simulink model "model"  (R2016a)
(part 10 of 11)

  548_CN_137197826_380000_CN_52983550_380000/LConn2 -- T_137197826_380000;220000;110000_Neuenhagen/LConn2 -- 517_CN_137197826_380000_CN_20562114_380000/LConn2 -- 495;_496_CN_137197826_380000_CN_22973070_380000/LConn2 -- 548_CN_137197826_380000_CN_23025610_380000/LConn2 -- 517_CN_137197826_380000_CN_29877599_380000/RConn2
  548_CN_137197826_380000_CN_52983550_380000/LConn3 -- T_137197826_380000;220000;110000_Neuenhagen/LConn3 -- 517_CN_137197826_380000_CN_20562114_380000/LConn3 -- 495;_496_CN_137197826_380000_CN_22973070_380000/LConn3 -- 548_CN_137197826_380000_CN_23025610_380000/LConn3 -- 517_CN_137197826_380000_CN_29877599_380000/RConn3
  T_52983550_380000;110000_Eisenhüttenstadt/LConn1 -- 548_CN_137197826_380000_CN_52983550_380000/RConn1
  T_52983550_380000;110000_Eisenhüttenstadt/LConn2 -- 548_CN_137197826_380000_CN_52983550_380000/RConn2
  T_52983550_380000;110000_Eisenhüttenstadt/LConn3 -- 548_CN_137197826_380000_CN_52983550_380000/RConn3
  548_CN_137197826_380000_CN_23025610_380000/RConn1 -- T_23025610_380000;110000_Umspannwerk_Preilack/LConn1 -- 561_CN_30164703_380000_CN_23025610_380000/LConn1 -- _CN_156683994_380000_CN_23025610_380000/LConn1 -- 559_CN_157328339_380000_CN_23025610_380000/LConn1 -- _CN_23025610_380000_CN11341038/LConn1
  548_CN_137197826_380000_CN_23025610_380000/RConn2 -- T_23025610_380000;110000_Umspannwerk_Preilack/LConn2 -- 561_CN_30164703_380000_CN_23025610_380000/LConn2 -- _CN_156683994_380000_CN_23025610_380000/LConn2 -- 559_CN_157328339_380000_CN_23025610_380000/LConn2 -- _CN_23025610_380000_CN11341038/LConn2
  548_CN_137197826_380000_CN_23025610_380000/RConn3 -- T_23025610_380000;110000_Umspannwerk_Preilack/LConn3 -- 561_CN_30164703_380000_CN_23025610_380000/LConn3 -- _CN_156683994_380000_CN_23025610_380000/LConn3 -- 559_CN_157328339_380000_CN_23025610_380000/LConn3 -- _CN_23025610_380000_CN11341038/LConn3
  T_20562114_380000;110000_Umspannwerk_Malchow/LConn1 -- 517_CN_137197826_380000_CN_20562114_380000/RConn1
  T_20562114_380000;110000_Umspannwerk_Malchow/LConn2 -- 517_CN_137197826_380000_CN_20562114_380000/RConn2
  T_20562114_380000;110000_Umspannwerk_Malchow/LConn3 -- 517_CN_137197826_380000_CN_20562114_380000/RConn3
  495;_496_CN_137197826_380000_CN_22973070_380000/RConn1 -- T_22973070_380000;220000;110000_Umspannwerk_Marzahn/LConn1 -- _CN_22973070_380000_CN_30954714_380000/LConn1
  495;_496_CN_137197826_380000_CN_22973070_380000/RConn2 -- T_22973070_380000;220000;110000_Umspannwerk_Marzahn/LConn2 -- _CN_22973070_380000_CN_30954714_380000/LConn2
  495;_496_CN_137197826_380000_CN_22973070_380000/RConn3 -- T_22973070_380000;220000;110000_Umspannwerk_Marzahn/LConn3 -- _CN_22973070_380000_CN_30954714_380000/LConn3
  526_CN_29331499_220000_CN_27149550_220000/LConn1 -- T_29331499_380000;220000;110000_Thyrow/RConn1 -- 302_CN_29331499_220000_CN_22973070_220000/LConn1 -- 302_CN_29331499_220000_CN_22973052_220000/LConn1
  526_CN_29331499_220000_CN_27149550_220000/LConn2 -- T_29331499_380000;220000;110000_Thyrow/RConn2 -- 302_CN_29331499_220000_CN_22973070_220000/LConn2 -- 302_CN_29331499_220000_CN_22973052_220000/LConn2
  526_CN_29331499_220000_CN_27149550_220000/LConn3 -- T_29331499_380000;220000;110000_Thyrow/RConn3 -- 302_CN_29331499_220000_CN_22973070_220000/LConn3 -- 302_CN_29331499_220000_CN_22973052_220000/LConn3
  526_CN_29331499_220000_CN_27149550_220000/RConn1 -- T_27149550_380000;220000;110000_Wustermark/RConn1 -- 294_CN_27149550_220000_CN215092049/RConn1 -- 294_CN_27149550_220000_CN_30309989_220000/LConn1 -- 324_CN_40621568_220000_CN_27149550_220000/LConn1
  526_CN_29331499_220000_CN_27149550_220000/RConn2 -- T_27149550_380000;220000;110000_Wustermark/RConn2 -- 294_CN_27149550_220000_CN215092049/RConn2 -- 294_CN_27149550_220000_CN_30309989_220000/LConn2 -- 324_CN_40621568_220000_CN_27149550_220000/LConn2
  526_CN_29331499_220000_CN_27149550_220000/RConn3 -- T_27149550_380000;220000;110000_Wustermark/RConn3 -- 294_CN_27149550_220000_CN215092049/RConn3 -- 294_CN_27149550_220000_CN_30309989_220000/LConn3 -- 324_CN_40621568_220000_CN_27149550_220000/LConn3
  302_CN_29331499_220000_CN_22973070_220000/RConn1 -- T_22973070_380000;220000;110000_Umspannwerk_Marzahn/RConn1 -- _CN_285823537_220000_CN_22973070_220000/LConn1
  302_CN_29331499_220000_CN_22973070_220000/RConn2 -- T_22973070_380000;220000;110000_Umspannwerk_Marzahn/RConn2 -- _CN_285823537_220000_CN_22973070_220000/LConn2
  302_CN_29331499_220000_CN_22973070_220000/RConn3 -- T_22973070_380000;220000;110000_Umspannwerk_Marzahn/RConn3 -- _CN_285823537_220000_CN_22973070_220000/LConn3
  T_22973052_220000;110000_Umspannwerk_Wuhlheide/LConn1 -- 302_CN_29331499_220000_CN_22973052_220000/RConn1
  T_22973052_220000;110000_Umspannwerk_Wuhlheide/LConn2 -- 302_CN_29331499_220000_CN_22973052_220000/RConn2
  T_22973052_220000;110000_Umspannwerk_Wuhlheide/LConn3 -- 302_CN_29331499_220000_CN_22973052_220000/RConn3
  T_29331499_380000;220000;110000_Thyrow/LConn1 -- 522_CN_29331499_380000_CN_27149550_380000/LConn1
  T_29331499_380000;220000;110000_Thyrow/LConn2 -- 522_CN_29331499_380000_CN_27149550_380000/LConn2
  T_29331499_380000;220000;110000_Thyrow/LConn3 -- 522_CN_29331499_380000_CN_27149550_380000/LConn3
  522_CN_29331499_380000_CN_27149550_380000/RConn1 -- T_27149550_380000;220000;110000_Wustermark/LConn1 -- 493_CN_26472665_380000_CN_27149550_380000/LConn1
  522_CN_29331499_380000_CN_27149550_380000/RConn2 -- T_27149550_380000;220000;110000_Wustermark/LConn2 -- 493_CN_26472665_380000_CN_27149550_380000/LConn2
  522_CN_29331499_380000_CN_27149550_380000/RConn3 -- T_27149550_380000;220000;110000_Wustermark/LConn3 -- 493_CN_26472665_380000_CN_27149550_380000/LConn3
  Helmstedt_380_kV_CN_26474759_380000_CN_24258096_380000/RConn1 -- T_26474759_380000;110000_Umspannwerk_Helmstedt/LConn1 -- Helmstedt_380_kV_CN_26474759_380000_CN_26472665_380000/LConn1 -- Leitung_3845_(System_301)_CN_26474759_380000_CN_199382606_380000/LConn1
  Helmstedt_380_kV_CN_26474759_380000_CN_24258096_380000/RConn2 -- T_26474759_380000;110000_Umspannwerk_Helmstedt/LConn2 -- Helmstedt_380_kV_CN_26474759_380000_CN_26472665_380000/LConn2 -- Leitung_3845_(System_301)_CN_26474759_380000_CN_199382606_380000/LConn2
  Helmstedt_380_kV_CN_26474759_380000_CN_24258096_380000/RConn3 -- T_26474759_380000;110000_Umspannwerk_Helmstedt/LConn3 -- Helmstedt_380_kV_CN_26474759_380000_CN_26472665_380000/LConn3 -- Leitung_3845_(System_301)_CN_26474759_380000_CN_199382606_380000/LConn3
  T_199382606__/LConn1 -- Leitung_3845_(System_301)_CN_26474759_380000_CN_199382606_380000/RConn1
  T_199382606__/LConn2 -- Leitung_3845_(System_301)_CN_26474759_380000_CN_199382606_380000/RConn2
  T_199382606__/LConn3 -- Leitung_3845_(System_301)_CN_26474759_380000_CN_199382606_380000/RConn3
  Helmstedt_380_kV_CN_26474759_380000_CN_26472665_380000/RConn1 -- T_26472665_380000;220000_Umspannwerk_Wolmirstedt/LConn1 -- 493_CN_26472665_380000_CN_30132758_380000/LConn1 -- 493_CN_26472665_380000_CN_27149550_380000/RConn1 -- 438_CN_26472665_380000_CN_156683994_380000/LConn1 -- 536_CN_26472665_380000_CN_32690742_380000/LConn1 -- 536_CN_26472665_380000_CN_29713902_380000/LConn1 -- 490_CN_26472665_380000_CN_33169401_380000/RConn1
  Helmstedt_380_kV_CN_26474759_380000_CN_26472665_380000/RConn2 -- T_26472665_380000;220000_Umspannwerk_Wolmirstedt/LConn2 -- 493_CN_26472665_380000_CN_30132758_380000/LConn2 -- 493_CN_26472665_380000_CN_27149550_380000/RConn2 -- 438_CN_26472665_380000_CN_156683994_380000/LConn2 -- 536_CN_26472665_380000_CN_32690742_380000/LConn2 -- 536_CN_26472665_380000_CN_29713902_380000/LConn2 -- 490_CN_26472665_380000_CN_33169401_380000/RConn2
  Helmstedt_380_kV_CN_26474759_380000_CN_26472665_380000/RConn3 -- T_26472665_380000;220000_Umspannwerk_Wolmirstedt/LConn3 -- 493_CN_26472665_380000_CN_30132758_380000/LConn3 -- 493_CN_26472665_380000_CN_27149550_380000/RConn3 -- 438_CN_26472665_380000_CN_156683994_380000/LConn3 -- 536_CN_26472665_380000_CN_32690742_380000/LConn3 -- 536_CN_26472665_380000_CN_29713902_380000/LConn3 -- 490_CN_26472665_380000_CN_33169401_380000/RConn3
  _CN_29344008_220000_CN_151765495_220000/RConn1 -- T_151765495_220000_Götzdorf/LConn1 -- _CN_151765495_220000_CN_229500139_220000/LConn1
  _CN_29344008_220000_CN_151765495_220000/RConn2 -- T_151765495_220000_Götzdorf/LConn2 -- _CN_151765495_220000_CN_229500139_220000/LConn2
  _CN_29344008_220000_CN_151765495_220000/RConn3 -- T_151765495_220000_Götzdorf/LConn3 -- _CN_151765495_220000_CN_229500139_220000/LConn3
  T_25306938_220000;110000_Kummerfeld/LConn1 -- _CN_29344008_220000_CN_25306938_220000/RConn1
  T_25306938_220000;110000_Kummerfeld/LConn2 -- _CN_29344008_220000_CN_25306938_220000/RConn2
  T_25306938_220000;110000_Kummerfeld/LConn3 -- _CN_29344008_220000_CN_25306938_220000/RConn3
  _CN_25557259_380000_CN_43688805_380000/LConn1 -- T_25557259__/LConn1 -- _CN_25557259_380000_CN_143854536_380000/LConn1 -- _CN_25557259_380000_CN_25557397_380000/LConn1 -- _CN_25557259_380000_CN_145002769_380000/LConn1 -- _CN_25557259_380000_CN_143903369_380000/LConn1 -- _CN_25557259_380000_CN_153328698_380000/LConn1 -- _CN_25557259_380000_CN89183108/LConn1
  _CN_25557259_380000_CN_43688805_380000/LConn2 -- T_25557259__/LConn2 -- _CN_25557259_380000_CN_143854536_380000/LConn2 -- _CN_25557259_380000_CN_25557397_380000/LConn2 -- _CN_25557259_380000_CN_145002769_380000/LConn2 -- _CN_25557259_380000_CN_143903369_380000/LConn2 -- _CN_25557259_380000_CN_153328698_380000/LConn2 -- _CN_25557259_380000_CN89183108/LConn2
  _CN_25557259_380000_CN_43688805_380000/LConn3 -- T_25557259__/LConn3 -- _CN_25557259_380000_CN_143854536_380000/LConn3 -- _CN_25557259_380000_CN_25557397_380000/LConn3 -- _CN_25557259_380000_CN_145002769_380000/LConn3 -- _CN_25557259_380000_CN_143903369_380000/LConn3 -- _CN_25557259_380000_CN_153328698_380000/LConn3 -- _CN_25557259_380000_CN89183108/LConn3
  _CN_25557259_380000_CN_43688805_380000/RConn1 -- T_43688805_380000;220000;110000_380kV_Umspannwerk_Pulverdingen/LConn1 -- Philippsburg___Pulverdingen_CN_43688805_380000_CN_254326606_380000/LConn1 -- Philippsburg___Pulverdingen_CN_43688805_380000_CN_154110135_380000/RConn1 -- 380_kV_CN_26260052_380000_CN_43688805_380000/LConn1 -- 2x_380_kV_CN_43688805_380000_CN_26814283_380000/LConn1
  _CN_25557259_380000_CN_43688805_380000/RConn2 -- T_43688805_380000;220000;110000_380kV_Umspannwerk_Pulverdingen/LConn2 -- Philippsburg___Pulverdingen_CN_43688805_380000_CN_254326606_380000/LConn2 -- Philippsburg___Pulverdingen_CN_43688805_380000_CN_154110135_380000/RConn2 -- 380_kV_CN_26260052_380000_CN_43688805_380000/LConn2 -- 2x_380_kV_CN_43688805_380000_CN_26814283_380000/LConn2
  _CN_25557259_380000_CN_43688805_380000/RConn3 -- T_43688805_380000;220000;110000_380kV_Umspannwerk_Pulverdingen/LConn3 -- Philippsburg___Pulverdingen_CN_43688805_380000_CN_254326606_380000/LConn3 -- Philippsburg___Pulverdingen_CN_43688805_380000_CN_154110135_380000/RConn3 -- 380_kV_CN_26260052_380000_CN_43688805_380000/LConn3 -- 2x_380_kV_CN_43688805_380000_CN_26814283_380000/LConn3
  _CN_25557259_380000_CN89183108/RConn1 -- G_89183108_Heizkraftwerk_Heilbronn/RConn1 -- _CN_25557397_220000_CN89183108/RConn1
  _CN_25557259_380000_CN89183108/RConn2 -- G_89183108_Heizkraftwerk_Heilbronn/RConn2 -- _CN_25557397_220000_CN89183108/RConn2
  _CN_25557259_380000_CN89183108/RConn3 -- G_89183108_Heizkraftwerk_Heilbronn/RConn3 -- _CN_25557397_220000_CN89183108/RConn3
  _CN_25557259_380000_CN_143854536_380000/RConn1 -- T_143854536_380000;110000_Umspannwerk_Kupferzell/LConn1 -- _CN_145002769_380000_CN_143854536_380000/LConn1 -- Goldshöfe___Kupferzell_CN_42050342_380000_CN_143854536_380000/RConn1
  _CN_25557259_380000_CN_143854536_380000/RConn2 -- T_143854536_380000;110000_Umspannwerk_Kupferzell/LConn2 -- _CN_145002769_380000_CN_143854536_380000/LConn2 -- Goldshöfe___Kupferzell_CN_42050342_380000_CN_143854536_380000/RConn2
  _CN_25557259_380000_CN_143854536_380000/RConn3 -- T_143854536_380000;110000_Umspannwerk_Kupferzell/LConn3 -- _CN_145002769_380000_CN_143854536_380000/LConn3 -- Goldshöfe___Kupferzell_CN_42050342_380000_CN_143854536_380000/RConn3
  T_25557397_380000;220000;110000_380_kV_Umspannwerk_Großgartach/LConn1 -- _CN_25557259_380000_CN_25557397_380000/RConn1
  T_25557397_380000;220000;110000_380_kV_Umspannwerk_Großgartach/LConn2 -- _CN_25557259_380000_CN_25557397_380000/RConn2
  T_25557397_380000;220000;110000_380_kV_Umspannwerk_Großgartach/LConn3 -- _CN_25557259_380000_CN_25557397_380000/RConn3
  _CN_25557259_380000_CN_145002769_380000/RConn1 -- T_145002769_380000;110000_Umspannwerk_Höpfingen/LConn1 -- _CN_145002769_380000_CN_108797675_380000/RConn1 -- _CN_145002769_380000_CN_143854536_380000/RConn1
  _CN_25557259_380000_CN_145002769_380000/RConn2 -- T_145002769_380000;110000_Umspannwerk_Höpfingen/LConn2 -- _CN_145002769_380000_CN_108797675_380000/RConn2 -- _CN_145002769_380000_CN_143854536_380000/RConn2
  _CN_25557259_380000_CN_145002769_380000/RConn3 -- T_145002769_380000;110000_Umspannwerk_Höpfingen/LConn3 -- _CN_145002769_380000_CN_108797675_380000/RConn3 -- _CN_145002769_380000_CN_143854536_380000/RConn3
  _CN_25557259_380000_CN_143903369_380000/RConn1 -- T_143903369_380000;220000;110000_Umspannwerk_Hüffenhardt/LConn1 -- Elsenz_CN_143903369_380000_CN_46584363_380000/LConn1 -- Elsenz_CN_143903369_380000_CN_154110135_380000/RConn1 -- Elsenz_CN_143903369_380000_CN_207248812_380000/LConn1
  _CN_25557259_380000_CN_143903369_380000/RConn2 -- T_143903369_380000;220000;110000_Umspannwerk_Hüffenhardt/LConn2 -- Elsenz_CN_143903369_380000_CN_46584363_380000/LConn2 -- Elsenz_CN_143903369_380000_CN_154110135_380000/RConn2 -- Elsenz_CN_143903369_380000_CN_207248812_380000/LConn2
  _CN_25557259_380000_CN_143903369_380000/RConn3 -- T_143903369_380000;220000;110000_Umspannwerk_Hüffenhardt/LConn3 -- Elsenz_CN_143903369_380000_CN_46584363_380000/LConn3 -- Elsenz_CN_143903369_380000_CN_154110135_380000/RConn3 -- Elsenz_CN_143903369_380000_CN_207248812_380000/LConn3
  _CN_25557259_380000_CN_153328698_380000/RConn1 -- T_153328698_380000_Gemeinschaftskraftwerk_Neckarwestheim_2/LConn1 -- _CN_147878692_380000_CN_153328698_380000/LConn1 -- _CN_153328698_380000_CN23547196/RConn1
  _CN_25557259_380000_CN_153328698_380000/RConn2 -- T_153328698_380000_Gemeinschaftskraftwerk_Neckarwestheim_2/LConn2 -- _CN_147878692_380000_CN_153328698_380000/LConn2 -- _CN_153328698_380000_CN23547196/RConn2
  _CN_25557259_380000_CN_153328698_380000/RConn3 -- T_153328698_380000_Gemeinschaftskraftwerk_Neckarwestheim_2/LConn3 -- _CN_147878692_380000_CN_153328698_380000/LConn3 -- _CN_153328698_380000_CN23547196/RConn3
  T_169244940_380000_Station_Kelsterbach/LConn1 -- _CN_169244940_380000_CN_55730023_380000/LConn1
  T_169244940_380000_Station_Kelsterbach/LConn2 -- _CN_169244940_380000_CN_55730023_380000/LConn2
  T_169244940_380000_Station_Kelsterbach/LConn3 -- _CN_169244940_380000_CN_55730023_380000/LConn3
  _CN_169244940_380000_CN_55730023_380000/RConn1 -- T_55730023_380000_Kabeleinführung_380_kV/LConn1 -- 2_x_380_kV;_3_x_220_kV_CN_23284340_380000_CN_55730023_380000/LConn1
  _CN_169244940_380000_CN_55730023_380000/RConn2 -- T_55730023_380000_Kabeleinführung_380_kV/LConn2 -- 2_x_380_kV;_3_x_220_kV_CN_23284340_380000_CN_55730023_380000/LConn2
  _CN_169244940_380000_CN_55730023_380000/RConn3 -- T_55730023_380000_Kabeleinführung_380_kV/LConn3 -- 2_x_380_kV;_3_x_220_kV_CN_23284340_380000_CN_55730023_380000/LConn3
  T_29417741_220000_Umspannwerk_Regensburg/LConn1 -- Regensburg___Schwandorf_CN_29417741_220000_CN_28956649_220000/RConn1
  T_29417741_220000_Umspannwerk_Regensburg/LConn2 -- Regensburg___Schwandorf_CN_29417741_220000_CN_28956649_220000/RConn2
  T_29417741_220000_Umspannwerk_Regensburg/LConn3 -- Regensburg___Schwandorf_CN_29417741_220000_CN_28956649_220000/RConn3
  501_CN_28729619_380000_CN_25526912_380000/LConn1 -- T_28729619_380000_Umspannwerk_Schönewalde/LConn1 -- 501_CN_28729619_380000_CN_156683994_380000/LConn1 -- 501_CN_28729619_380000_CN_29713902_380000/LConn1
  501_CN_28729619_380000_CN_25526912_380000/LConn2 -- T_28729619_380000_Umspannwerk_Schönewalde/LConn2 -- 501_CN_28729619_380000_CN_156683994_380000/LConn2 -- 501_CN_28729619_380000_CN_29713902_380000/LConn2
  501_CN_28729619_380000_CN_25526912_380000/LConn3 -- T_28729619_380000_Umspannwerk_Schönewalde/LConn3 -- 501_CN_28729619_380000_CN_156683994_380000/LConn3 -- 501_CN_28729619_380000_CN_29713902_380000/LConn3
  T_25526912_380000;110000_Umspannwerk_Marke/LConn1 -- 501_CN_28729619_380000_CN_25526912_380000/RConn1
  T_25526912_380000;110000_Umspannwerk_Marke/LConn2 -- 501_CN_28729619_380000_CN_25526912_380000/RConn2
  T_25526912_380000;110000_Umspannwerk_Marke/LConn3 -- 501_CN_28729619_380000_CN_25526912_380000/RConn3
  501_CN_28729619_380000_CN_29713902_380000/RConn1 -- T_29713902_380000;110000_Umspannwerk_Lauchstädt/LConn1 -- _CN_29713902_380000_CN218161891/LConn1 -- _CN_143882655_380000_CN_29713902_380000/RConn1 -- 536_CN_26472665_380000_CN_29713902_380000/RConn1
  501_CN_28729619_380000_CN_29713902_380000/RConn2 -- T_29713902_380000;110000_Umspannwerk_Lauchstädt/LConn2 -- _CN_29713902_380000_CN218161891/LConn2 -- _CN_143882655_380000_CN_29713902_380000/RConn2 -- 536_CN_26472665_380000_CN_29713902_380000/RConn2
  501_CN_28729619_380000_CN_29713902_380000/RConn3 -- T_29713902_380000;110000_Umspannwerk_Lauchstädt/LConn3 -- _CN_29713902_380000_CN218161891/LConn3 -- _CN_143882655_380000_CN_29713902_380000/RConn3 -- 536_CN_26472665_380000_CN_29713902_380000/RConn3
  501_CN_28729619_380000_CN_156683994_380000/RConn1 -- T_156683994_380000;110000_Umspannwerk_Ragow/LConn1 -- _CN_156683994_380000_CN_23025610_380000/RConn1 -- 438_CN_26472665_380000_CN_156683994_380000/RConn1 -- 561_Streumen_CN_156683994_380000_CN_157328339_380000/LConn1
  501_CN_28729619_380000_CN_156683994_380000/RConn2 -- T_156683994_380000;110000_Umspannwerk_Ragow/LConn2 -- _CN_156683994_380000_CN_23025610_380000/RConn2 -- 438_CN_26472665_380000_CN_156683994_380000/RConn2 -- 561_Streumen_CN_156683994_380000_CN_157328339_380000/LConn2
  501_CN_28729619_380000_CN_156683994_380000/RConn3 -- T_156683994_380000;110000_Umspannwerk_Ragow/LConn3 -- _CN_156683994_380000_CN_23025610_380000/RConn3 -- 438_CN_26472665_380000_CN_156683994_380000/RConn3 -- 561_Streumen_CN_156683994_380000_CN_157328339_380000/LConn3
  T_53378027_380000;110000_Umspannwerk_Lechhausen;_Übernahmestation_Lechhausen/LConn1 -- _CN_30613895_380000_CN_53378027_380000/RConn1
  T_53378027_380000;110000_Umspannwerk_Lechhausen;_Übernahmestation_Lechhausen/LConn2 -- _CN_30613895_380000_CN_53378027_380000/RConn2
  T_53378027_380000;110000_Umspannwerk_Lechhausen;_Übernahmestation_Lechhausen/LConn3 -- _CN_30613895_380000_CN_53378027_380000/RConn3
  _CN_30613895_380000_CN_24652261_380000/RConn1 -- T_24652261_380000_Station_Meitingen/LConn1 -- Meitingen_Nord;_Süd_CN_24652261_380000_CN_85523877_380000/RConn1 -- Meitingen_Nord;_Süd_CN_24652261_380000_CN_88945213_380000/LConn1 -- _CN_24652261_380000_CN_76246159_380000/LConn1 -- MEI_OBA_CN_24652261_380000_CN_18629425_380000/RConn1
  _CN_30613895_380000_CN_24652261_380000/RConn2 -- T_24652261_380000_Station_Meitingen/LConn2 -- Meitingen_Nord;_Süd_CN_24652261_380000_CN_85523877_380000/RConn2 -- Meitingen_Nord;_Süd_CN_24652261_380000_CN_88945213_380000/LConn2 -- _CN_24652261_380000_CN_76246159_380000/LConn2 -- MEI_OBA_CN_24652261_380000_CN_18629425_380000/RConn2
  _CN_30613895_380000_CN_24652261_380000/RConn3 -- T_24652261_380000_Station_Meitingen/LConn3 -- Meitingen_Nord;_Süd_CN_24652261_380000_CN_85523877_380000/RConn3 -- Meitingen_Nord;_Süd_CN_24652261_380000_CN_88945213_380000/LConn3 -- _CN_24652261_380000_CN_76246159_380000/LConn3 -- MEI_OBA_CN_24652261_380000_CN_18629425_380000/RConn3
  380_kV_Gilzem_Ost;_Uchtelfangen_Ost_CN_42097854_380000_CN_54359256_380000/LConn1 -- T_42097854_380000;110000_Station_Osburg/LConn1 -- 380_kV_Gilzem_Ost;_Uchtelfangen_Ost_CN_42097854_380000_CN_151967290_380000/LConn1
  380_kV_Gilzem_Ost;_Uchtelfangen_Ost_CN_42097854_380000_CN_54359256_380000/LConn2 -- T_42097854_380000;110000_Station_Osburg/LConn2 -- 380_kV_Gilzem_Ost;_Uchtelfangen_Ost_CN_42097854_380000_CN_151967290_380000/LConn2
  380_kV_Gilzem_Ost;_Uchtelfangen_Ost_CN_42097854_380000_CN_54359256_380000/LConn3 -- T_42097854_380000;110000_Station_Osburg/LConn3 -- 380_kV_Gilzem_Ost;_Uchtelfangen_Ost_CN_42097854_380000_CN_151967290_380000/LConn3
  380_kV_Gilzem_Ost;_Uchtelfangen_Ost_CN_42097854_380000_CN_54359256_380000/RConn1 -- T_54359256_380000;220000;110000_Umspannwerk_Uchtelfangen/LConn1 -- _CN_54359256_380000_CN115145869/LConn1 -- _CN_152261133_380000_CN_54359256_380000/RConn1
  380_kV_Gilzem_Ost;_Uchtelfangen_Ost_CN_42097854_380000_CN_54359256_380000/RConn2 -- T_54359256_380000;220000;110000_Umspannwerk_Uchtelfangen/LConn2 -- _CN_54359256_380000_CN115145869/LConn2 -- _CN_152261133_380000_CN_54359256_380000/RConn2
  380_kV_Gilzem_Ost;_Uchtelfangen_Ost_CN_42097854_380000_CN_54359256_380000/RConn3 -- T_54359256_380000;220000;110000_Umspannwerk_Uchtelfangen/LConn3 -- _CN_54359256_380000_CN115145869/LConn3 -- _CN_152261133_380000_CN_54359256_380000/RConn3
  380_kV_Gilzem_Ost;_Uchtelfangen_Ost_CN_42097854_380000_CN_151967290_380000/RConn1 -- T_151967290_380000;220000;110000_Station_Niederstedem/LConn1 -- _CN_151967290_380000_CN_32675761_380000/LConn1 -- _CN_151967290_380000_CN_26593929_380000/RConn1
  380_kV_Gilzem_Ost;_Uchtelfangen_Ost_CN_42097854_380000_CN_151967290_380000/RConn2 -- T_151967290_380000;220000;110000_Station_Niederstedem/LConn2 -- _CN_151967290_380000_CN_32675761_380000/LConn2 -- _CN_151967290_380000_CN_26593929_380000/RConn2
  380_kV_Gilzem_Ost;_Uchtelfangen_Ost_CN_42097854_380000_CN_151967290_380000/RConn3 -- T_151967290_380000;220000;110000_Station_Niederstedem/LConn3 -- _CN_151967290_380000_CN_32675761_380000/LConn3 -- _CN_151967290_380000_CN_26593929_380000/RConn3
  220kV_Welper_Ost+ANK_CN_156973363_220000_CN_63114179_220000/LConn1 -- T_156973363_220000_Station_Welper/LConn1 -- 220kV_Welper_Ost+ANK_CN_156973363_220000_CN_86163350_220000/LConn1 -- 220kV_Welper_Ost+ANK_CN_156973363_220000_CN_68549340_220000/RConn1
  220kV_Welper_Ost+ANK_CN_156973363_220000_CN_63114179_220000/LConn2 -- T_156973363_220000_Station_Welper/LConn2 -- 220kV_Welper_Ost+ANK_CN_156973363_220000_CN_86163350_220000/LConn2 -- 220kV_Welper_Ost+ANK_CN_156973363_220000_CN_68549340_220000/RConn2
  220kV_Welper_Ost+ANK_CN_156973363_220000_CN_63114179_220000/LConn3 -- T_156973363_220000_Station_Welper/LConn3 -- 220kV_Welper_Ost+ANK_CN_156973363_220000_CN_86163350_220000/LConn3 -- 220kV_Welper_Ost+ANK_CN_156973363_220000_CN_68549340_220000/RConn3
  T_63114179_380000;220000;110000_Station_Hattingen/RConn1 -- 220kV_Welper_Ost+ANK_CN_156973363_220000_CN_63114179_220000/RConn1
  T_63114179_380000;220000;110000_Station_Hattingen/RConn2 -- 220kV_Welper_Ost+ANK_CN_156973363_220000_CN_63114179_220000/RConn2
  T_63114179_380000;220000;110000_Station_Hattingen/RConn3 -- 220kV_Welper_Ost+ANK_CN_156973363_220000_CN_63114179_220000/RConn3
  T_86163350_220000_UW_Stahlwerk_ThyssenKrupp_Nirosta/LConn1 -- 220kV_Welper_Ost+ANK_CN_156973363_220000_CN_86163350_220000/RConn1
  T_86163350_220000_UW_Stahlwerk_ThyssenKrupp_Nirosta/LConn2 -- 220kV_Welper_Ost+ANK_CN_156973363_220000_CN_86163350_220000/RConn2
  T_86163350_220000_UW_Stahlwerk_ThyssenKrupp_Nirosta/LConn3 -- 220kV_Welper_Ost+ANK_CN_156973363_220000_CN_86163350_220000/RConn3
  T_153334076__/LConn1 -- _CN_153334076_220000_CN23547196/RConn1
  T_153334076__/LConn2 -- _CN_153334076_220000_CN23547196/RConn2
  T_153334076__/LConn3 -- _CN_153334076_220000_CN23547196/RConn3
  329_CN_35102433_220000_CN_26472665_220000/LConn1 -- T_35102433_220000;110000_Magdeburg_(50Hertz)/LConn1 -- 335_CN_35102433_220000_CN_35137205_220000/LConn1
  329_CN_35102433_220000_CN_26472665_220000/LConn2 -- T_35102433_220000;110000_Magdeburg_(50Hertz)/LConn2 -- 335_CN_35102433_220000_CN_35137205_220000/LConn2
  329_CN_35102433_220000_CN_26472665_220000/LConn3 -- T_35102433_220000;110000_Magdeburg_(50Hertz)/LConn3 -- 335_CN_35102433_220000_CN_35137205_220000/LConn3
  329_CN_35102433_220000_CN_26472665_220000/RConn1 -- T_26472665_380000;220000_Umspannwerk_Wolmirstedt/RConn1 -- 344_CN_26472665_220000_CN_35137205_220000/LConn1 -- L_26472665/LConn1
  329_CN_35102433_220000_CN_26472665_220000/RConn2 -- T_26472665_380000;220000_Umspannwerk_Wolmirstedt/RConn2 -- 344_CN_26472665_220000_CN_35137205_220000/LConn2 -- L_26472665/LConn2
  329_CN_35102433_220000_CN_26472665_220000/RConn3 -- T_26472665_380000;220000_Umspannwerk_Wolmirstedt/RConn3 -- 344_CN_26472665_220000_CN_35137205_220000/LConn3 -- L_26472665/LConn3
  335_CN_35102433_220000_CN_35137205_220000/RConn1 -- T_35137205_220000;110000_Umspannwerk_Förderstedt/LConn1 -- 344_CN_26472665_220000_CN_35137205_220000/RConn1
  335_CN_35102433_220000_CN_35137205_220000/RConn2 -- T_35137205_220000;110000_Umspannwerk_Förderstedt/LConn2 -- 344_CN_26472665_220000_CN_35137205_220000/RConn2
  335_CN_35102433_220000_CN_35137205_220000/RConn3 -- T_35137205_220000;110000_Umspannwerk_Förderstedt/LConn3 -- 344_CN_26472665_220000_CN_35137205_220000/RConn3
  _CN_91086220_220000_CN_24976300_220000/LConn1 -- T_91086220_220000_Umspannwerk_Simbach/LConn1 -- _CN_91086220_220000_CN_77694901_220000/LConn1 -- _CN_91086220_220000_CN167578660/RConn1
  _CN_91086220_220000_CN_24976300_220000/LConn2 -- T_91086220_220000_Umspannwerk_Simbach/LConn2 -- _CN_91086220_220000_CN_77694901_220000/LConn2 -- _CN_91086220_220000_CN167578660/RConn2
  _CN_91086220_220000_CN_24976300_220000/LConn3 -- T_91086220_220000_Umspannwerk_Simbach/LConn3 -- _CN_91086220_220000_CN_77694901_220000/LConn3 -- _CN_91086220_220000_CN167578660/RConn3
  _CN_91086220_220000_CN_24976300_220000/RConn1 -- T_24976300_380000;220000;110000_Umspannwerk_Pleinting/RConn1 -- Pleinting___Schwandorf_CN_24976300_220000_CN_28956649_220000/RConn1
  _CN_91086220_220000_CN_24976300_220000/RConn2 -- T_24976300_380000;220000;110000_Umspannwerk_Pleinting/RConn2 -- Pleinting___Schwandorf_CN_24976300_220000_CN_28956649_220000/RConn2
  _CN_91086220_220000_CN_24976300_220000/RConn3 -- T_24976300_380000;220000;110000_Umspannwerk_Pleinting/RConn3 -- Pleinting___Schwandorf_CN_24976300_220000_CN_28956649_220000/RConn3
  _CN_91086220_220000_CN_77694901_220000/RConn1 -- T_77694901_220000;110000_Umspannwerk_Altheim/LConn1 -- Altheim___Sittling_CN_24759324_220000_CN_77694901_220000/LConn1
  _CN_91086220_220000_CN_77694901_220000/RConn2 -- T_77694901_220000;110000_Umspannwerk_Altheim/LConn2 -- Altheim___Sittling_CN_24759324_220000_CN_77694901_220000/LConn2
  _CN_91086220_220000_CN_77694901_220000/RConn3 -- T_77694901_220000;110000_Umspannwerk_Altheim/LConn3 -- Altheim___Sittling_CN_24759324_220000_CN_77694901_220000/LConn3
  _CN_152924498_220000_CN152506744/RConn1 -- G_152506744_Großkraftwerk_Mannheim/RConn1 -- _CN_163093653_220000_CN152506744/LConn1
  _CN_152924498_220000_CN152506744/RConn2 -- G_152506744_Großkraftwerk_Mannheim/RConn2 -- _CN_163093653_220000_CN152506744/LConn2
  _CN_152924498_220000_CN152506744/RConn3 -- G_152506744_Großkraftwerk_Mannheim/RConn3 -- _CN_163093653_220000_CN152506744/LConn3
  220kV_Fichtenhain_West+Utfort_West_CN_93278553_220000_CN_24815262_220000/LConn1 -- T_93278553_220000;110000_Station_Edelstahl_Krefeld/LConn1 -- 220kV_Fichtenhain_West+Utfort_West_CN_93278553_220000_CN_24799890_220000/RConn1 -- 220kV_Fichtenhain_West+Utfort_West_CN_93278553_220000_CN_23380800_220000/LConn1 -- 220kV_Fichtenhain_West+Utfort_West_CN_93278553_220000_CN92877616/LConn1 -- 220kV_Fichtenhain_West+Utfort_West_CN_93278553_220000_CN_91854336_220000/RConn1 -- 220kV_Fichtenhain_West+Utfort_West_CN_93278553_220000_CN_24479984_220000/LConn1
  220kV_Fichtenhain_West+Utfort_West_CN_93278553_220000_CN_24815262_220000/LConn2 -- T_93278553_220000;110000_Station_Edelstahl_Krefeld/LConn2 -- 220kV_Fichtenhain_West+Utfort_West_CN_93278553_220000_CN_24799890_220000/RConn2 -- 220kV_Fichtenhain_West+Utfort_West_CN_93278553_220000_CN_23380800_220000/LConn2 -- 220kV_Fichtenhain_West+Utfort_West_CN_93278553_220000_CN92877616/LConn2 -- 220kV_Fichtenhain_West+Utfort_West_CN_93278553_220000_CN_91854336_220000/RConn2 -- 220kV_Fichtenhain_West+Utfort_West_CN_93278553_220000_CN_24479984_220000/LConn2
  220kV_Fichtenhain_West+Utfort_West_CN_93278553_220000_CN_24815262_220000/LConn3 -- T_93278553_220000;110000_Station_Edelstahl_Krefeld/LConn3 -- 220kV_Fichtenhain_West+Utfort_West_CN_93278553_220000_CN_24799890_220000/RConn3 -- 220kV_Fichtenhain_West+Utfort_West_CN_93278553_220000_CN_23380800_220000/LConn3 -- 220kV_Fichtenhain_West+Utfort_West_CN_93278553_220000_CN92877616/LConn3 -- 220kV_Fichtenhain_West+Utfort_West_CN_93278553_220000_CN_91854336_220000/RConn3 -- 220kV_Fichtenhain_West+Utfort_West_CN_93278553_220000_CN_24479984_220000/LConn3
  T_24815262_380000;220000;110000_Station_Dülken/LConn1 -- 220kV_Fichtenhain_West+Utfort_West_CN_93278553_220000_CN_24815262_220000/RConn1
  T_24815262_380000;220000;110000_Station_Dülken/LConn2 -- 220kV_Fichtenhain_West+Utfort_West_CN_93278553_220000_CN_24815262_220000/RConn2
  T_24815262_380000;220000;110000_Station_Dülken/LConn3 -- 220kV_Fichtenhain_West+Utfort_West_CN_93278553_220000_CN_24815262_220000/RConn3
  220kV_Fichtenhain_West+Utfort_West_CN_93278553_220000_CN_23380800_220000/RConn1 -- T_23380800_380000;220000;110000_Station_Utfort/RConn1 -- 220kV_Wesel_Ost_CN_24462426_220000_CN_23380800_220000/RConn1
  220kV_Fichtenhain_West+Utfort_West_CN_93278553_220000_CN_23380800_220000/RConn2 -- T_23380800_380000;220000;110000_Station_Utfort/RConn2 -- 220kV_Wesel_Ost_CN_24462426_220000_CN_23380800_220000/RConn2
  220kV_Fichtenhain_West+Utfort_West_CN_93278553_220000_CN_23380800_220000/RConn3 -- T_23380800_380000;220000;110000_Station_Utfort/RConn3 -- 220kV_Wesel_Ost_CN_24462426_220000_CN_23380800_220000/RConn3
  220kV_Fichtenhain_West+Utfort_West_CN_93278553_220000_CN92877616/RConn1 -- G_92877616_Kraftwerk_Huckingen/RConn1 -- _CN_92877610_220000_CN92877616/LConn1 -- _CN_92877635_220000_CN92877616/LConn1
  220kV_Fichtenhain_West+Utfort_West_CN_93278553_220000_CN92877616/RConn2 -- G_92877616_Kraftwerk_Huckingen/RConn2 -- _CN_92877610_220000_CN92877616/LConn2 -- _CN_92877635_220000_CN92877616/LConn2
  220kV_Fichtenhain_West+Utfort_West_CN_93278553_220000_CN92877616/RConn3 -- G_92877616_Kraftwerk_Huckingen/RConn3 -- _CN_92877610_220000_CN92877616/LConn3 -- _CN_92877635_220000_CN92877616/LConn3
  T_24479984_220000;110000_Uerdingen/LConn1 -- 220kV_Fichtenhain_West+Utfort_West_CN_93278553_220000_CN_24479984_220000/RConn1
  T_24479984_220000;110000_Uerdingen/LConn2 -- 220kV_Fichtenhain_West+Utfort_West_CN_93278553_220000_CN_24479984_220000/RConn2
  T_24479984_220000;110000_Uerdingen/LConn3 -- 220kV_Fichtenhain_West+Utfort_West_CN_93278553_220000_CN_24479984_220000/RConn3
  T_74893659_380000;110000_HGÜ_Baltic_Cable___Stromrichterstation_Herrenwyk/LConn1 -- _CN_74893659_380000_CN_74893662_380000/LConn1
  T_74893659_380000;110000_HGÜ_Baltic_Cable___Stromrichterstation_Herrenwyk/LConn2 -- _CN_74893659_380000_CN_74893662_380000/LConn2
  T_74893659_380000;110000_HGÜ_Baltic_Cable___Stromrichterstation_Herrenwyk/LConn3 -- _CN_74893659_380000_CN_74893662_380000/LConn3
  T_74893662_380000;220000;110000_Umspannwerk_Siems/LConn1 -- _CN_74893659_380000_CN_74893662_380000/RConn1
  T_74893662_380000;220000;110000_Umspannwerk_Siems/LConn2 -- _CN_74893659_380000_CN_74893662_380000/RConn2
  T_74893662_380000;220000;110000_Umspannwerk_Siems/LConn3 -- _CN_74893659_380000_CN_74893662_380000/RConn3
  Scholven_C_CN_38584673_220000_CN22943608/RConn1 -- G_22943608_Kraftwerk_Scholven/RConn1 -- 220kV_Scholven_E_CN_23022100_220000_CN22943608/RConn1 -- 380kV_Scholven_B_CN_23022100_380000_CN22943608/RConn1
  Scholven_C_CN_38584673_220000_CN22943608/RConn2 -- G_22943608_Kraftwerk_Scholven/RConn2 -- 220kV_Scholven_E_CN_23022100_220000_CN22943608/RConn2 -- 380kV_Scholven_B_CN_23022100_380000_CN22943608/RConn2
  Scholven_C_CN_38584673_220000_CN22943608/RConn3 -- G_22943608_Kraftwerk_Scholven/RConn3 -- 220kV_Scholven_E_CN_23022100_220000_CN22943608/RConn3 -- 380kV_Scholven_B_CN_23022100_380000_CN22943608/RConn3
  T_89352550_380000;220000;110000_Bexbach_Kraftwerk/LConn1 -- _CN_89352550_380000_CN28051874/LConn1
  T_89352550_380000;220000;110000_Bexbach_Kraftwerk/LConn2 -- _CN_89352550_380000_CN28051874/LConn2
  T_89352550_380000;220000;110000_Bexbach_Kraftwerk/LConn3 -- _CN_89352550_380000_CN28051874/LConn3
  _CN_89352550_380000_CN28051874/RConn1 -- G_28051874_Kraftwerk_Bexbach/RConn1 -- _CN_152018146_380000_CN28051874/LConn1
  _CN_89352550_380000_CN28051874/RConn2 -- G_28051874_Kraftwerk_Bexbach/RConn2 -- _CN_152018146_380000_CN28051874/LConn2
  _CN_89352550_380000_CN28051874/RConn3 -- G_28051874_Kraftwerk_Bexbach/RConn3 -- _CN_152018146_380000_CN28051874/LConn3
  220_kV_Bigge_Ost|West_CN_22761839_220000_CN_156398578_220000/RConn1 -- T_156398578__Station_Ronsdorf/LConn1 -- 220kV_Bixterheide_Nord+Bigge_Ost_CN_51940126_220000_CN_156398578_220000/LConn1
  220_kV_Bigge_Ost|West_CN_22761839_220000_CN_156398578_220000/RConn2 -- T_156398578__Station_Ronsdorf/LConn2 -- 220kV_Bixterheide_Nord+Bigge_Ost_CN_51940126_220000_CN_156398578_220000/LConn2
  220_kV_Bigge_Ost|West_CN_22761839_220000_CN_156398578_220000/RConn3 -- T_156398578__Station_Ronsdorf/LConn3 -- 220kV_Bixterheide_Nord+Bigge_Ost_CN_51940126_220000_CN_156398578_220000/LConn3
  T_22761692_220000;110000_UW_Fühlingen/LConn1 -- 220_kV_Niederaußem_4d;_Wiesdorf_Ltg__CN_22761839_220000_CN_22761692_220000/RConn1
  T_22761692_220000;110000_UW_Fühlingen/LConn2 -- 220_kV_Niederaußem_4d;_Wiesdorf_Ltg__CN_22761839_220000_CN_22761692_220000/RConn2
  T_22761692_220000;110000_UW_Fühlingen/LConn3 -- 220_kV_Niederaußem_4d;_Wiesdorf_Ltg__CN_22761839_220000_CN_22761692_220000/RConn3
  220_kV_Niederaußem_4d;_Wiesdorf_Ltg__CN_22761839_220000_CN_24839976_220000/RConn1 -- T_24839976_380000;220000_Umspannwerk_Rommerskirchen/RConn1 -- 220_kV_Rommerskirchen_Ost_CN_24839976_220000_CN_23084554_220000/LConn1 -- 220_kV_Frixheim_Nord|Süd_CN_24839976_220000_CN_27919734_220000/LConn1 -- L_24839976/LConn1
  220_kV_Niederaußem_4d;_Wiesdorf_Ltg__CN_22761839_220000_CN_24839976_220000/RConn2 -- T_24839976_380000;220000_Umspannwerk_Rommerskirchen/RConn2 -- 220_kV_Rommerskirchen_Ost_CN_24839976_220000_CN_23084554_220000/LConn2 -- 220_kV_Frixheim_Nord|Süd_CN_24839976_220000_CN_27919734_220000/LConn2 -- L_24839976/LConn2
  220_kV_Niederaußem_4d;_Wiesdorf_Ltg__CN_22761839_220000_CN_24839976_220000/RConn3 -- T_24839976_380000;220000_Umspannwerk_Rommerskirchen/RConn3 -- 220_kV_Rommerskirchen_Ost_CN_24839976_220000_CN_23084554_220000/LConn3 -- 220_kV_Frixheim_Nord|Süd_CN_24839976_220000_CN_27919734_220000/LConn3 -- L_24839976/LConn3
  220_kV_Niederaußem_4d;_Wiesdorf_Ltg__CN_22761839_220000_CN-1726424/RConn1 -- G_-1726424_RWE_Kraftwerk_Niederaußem/RConn1 -- 220_kV_Niederaußem_3c_CN_32993727_220000_CN-1726424/LConn1 -- _CN_24839976_380000_CN-1726424/RConn1
  220_kV_Niederaußem_4d;_Wiesdorf_Ltg__CN_22761839_220000_CN-1726424/RConn2 -- G_-1726424_RWE_Kraftwerk_Niederaußem/RConn2 -- 220_kV_Niederaußem_3c_CN_32993727_220000_CN-1726424/LConn2 -- _CN_24839976_380000_CN-1726424/RConn2
  220_kV_Niederaußem_4d;_Wiesdorf_Ltg__CN_22761839_220000_CN-1726424/RConn3 -- G_-1726424_RWE_Kraftwerk_Niederaußem/RConn3 -- 220_kV_Niederaußem_3c_CN_32993727_220000_CN-1726424/LConn3 -- _CN_24839976_380000_CN-1726424/RConn3
  T_22764922_220000;110000_Station_Dhünnaue/LConn1 -- 220_kV_Niederaußem_4d;_Wiesdorf_Ltg__CN_22761839_220000_CN_22764922_220000/RConn1
  T_22764922_220000;110000_Station_Dhünnaue/LConn2 -- 220_kV_Niederaußem_4d;_Wiesdorf_Ltg__CN_22761839_220000_CN_22764922_220000/RConn2
  T_22764922_220000;110000_Station_Dhünnaue/LConn3 -- 220_kV_Niederaußem_4d;_Wiesdorf_Ltg__CN_22761839_220000_CN_22764922_220000/RConn3
  380_kV_Neurath_2b;_Oerkhaus_Ost_CN_22761839_380000_CN_49577448_380000/RConn1 -- T_49577448_380000;220000_Station_Sankt_Peter_380_kV/LConn1 -- 380kV_Knechtsteden_West_CN_77179271_380000_CN_49577448_380000/LConn1
  380_kV_Neurath_2b;_Oerkhaus_Ost_CN_22761839_380000_CN_49577448_380000/RConn2 -- T_49577448_380000;220000_Station_Sankt_Peter_380_kV/LConn2 -- 380kV_Knechtsteden_West_CN_77179271_380000_CN_49577448_380000/LConn2
  380_kV_Neurath_2b;_Oerkhaus_Ost_CN_22761839_380000_CN_49577448_380000/RConn3 -- T_49577448_380000;220000_Station_Sankt_Peter_380_kV/LConn3 -- 380kV_Knechtsteden_West_CN_77179271_380000_CN_49577448_380000/LConn3
  T_106096507_380000;110000_Station_Ohligs/LConn1 -- 380_kV_Neurath_2b;_Oerkhaus_Ost_CN_22761839_380000_CN_106096507_380000/RConn1
  T_106096507_380000;110000_Station_Ohligs/LConn2 -- 380_kV_Neurath_2b;_Oerkhaus_Ost_CN_22761839_380000_CN_106096507_380000/RConn2
  T_106096507_380000;110000_Station_Ohligs/LConn3 -- 380_kV_Neurath_2b;_Oerkhaus_Ost_CN_22761839_380000_CN_106096507_380000/RConn3
  380kV_Sauerland_Süd_CN_42799487_380000_CN_42488850_380000/RConn1 -- T_42799487_380000;110000_Station_Arpe/LConn1 -- 380kV_Sauerland_Süd_CN_42799487_380000_CN_42797575_380000/LConn1
  380kV_Sauerland_Süd_CN_42799487_380000_CN_42488850_380000/RConn2 -- T_42799487_380000;110000_Station_Arpe/LConn2 -- 380kV_Sauerland_Süd_CN_42799487_380000_CN_42797575_380000/LConn2
  380kV_Sauerland_Süd_CN_42799487_380000_CN_42488850_380000/RConn3 -- T_42799487_380000;110000_Station_Arpe/LConn3 -- 380kV_Sauerland_Süd_CN_42799487_380000_CN_42797575_380000/LConn3
  380kV_Sauerland_Süd_CN_42799487_380000_CN_42797575_380000/RConn1 -- T_42797575_380000;110000_Station_Nehden/LConn1 -- 380kV_Twistetal_Ost_3_CN_42797575_380000_CN_41232144_380000/LConn1 -- 380kV_Twistetal_Ost_3_CN_42797575_380000_CN_25943440_380000/LConn1
  380kV_Sauerland_Süd_CN_42799487_380000_CN_42797575_380000/RConn2 -- T_42797575_380000;110000_Station_Nehden/LConn2 -- 380kV_Twistetal_Ost_3_CN_42797575_380000_CN_41232144_380000/LConn2 -- 380kV_Twistetal_Ost_3_CN_42797575_380000_CN_25943440_380000/LConn2
  380kV_Sauerland_Süd_CN_42799487_380000_CN_42797575_380000/RConn3 -- T_42797575_380000;110000_Station_Nehden/LConn3 -- 380kV_Twistetal_Ost_3_CN_42797575_380000_CN_41232144_380000/LConn3 -- 380kV_Twistetal_Ost_3_CN_42797575_380000_CN_25943440_380000/LConn3
  380kV_Knechtsteden_West_CN_77179271_380000_CN_24839976_380000/RConn1 -- T_77179271_380000_Station_Osterath/LConn1 -- 380kV_Meerbusch_West_CN_77179271_380000_CN_25044557_380000/LConn1 -- 380kV_Knechtsteden_West_CN_77179271_380000_CN_49577448_380000/RConn1 -- 380kV_Knechtsteden_West_CN_77179271_380000_CN31783693/LConn1 -- 380kV_Knechtsteden_West_CN_77179271_380000_CN_207488608_380000/LConn1 -- 380kV_Meerbusch_West_CN_77179271_380000_CN_23380800_380000/LConn1
  380kV_Knechtsteden_West_CN_77179271_380000_CN_24839976_380000/RConn2 -- T_77179271_380000_Station_Osterath/LConn2 -- 380kV_Meerbusch_West_CN_77179271_380000_CN_25044557_380000/LConn2 -- 380kV_Knechtsteden_West_CN_77179271_380000_CN_49577448_380000/RConn2 -- 380kV_Knechtsteden_West_CN_77179271_380000_CN31783693/LConn2 -- 380kV_Knechtsteden_West_CN_77179271_380000_CN_207488608_380000/LConn2 -- 380kV_Meerbusch_West_CN_77179271_380000_CN_23380800_380000/LConn2
  380kV_Knechtsteden_West_CN_77179271_380000_CN_24839976_380000/RConn3 -- T_77179271_380000_Station_Osterath/LConn3 -- 380kV_Meerbusch_West_CN_77179271_380000_CN_25044557_380000/LConn3 -- 380kV_Knechtsteden_West_CN_77179271_380000_CN_49577448_380000/RConn3 -- 380kV_Knechtsteden_West_CN_77179271_380000_CN31783693/LConn3 -- 380kV_Knechtsteden_West_CN_77179271_380000_CN_207488608_380000/LConn3 -- 380kV_Meerbusch_West_CN_77179271_380000_CN_23380800_380000/LConn3
  380kV_Knechtsteden_West_CN_77179271_380000_CN31783693/RConn1 -- G_31783693_RWE_Kraftwerk_Neurath/RConn1 -- 220_kV_Neurath_1a_CN_27919734_220000_CN31783693/LConn1
  380kV_Knechtsteden_West_CN_77179271_380000_CN31783693/RConn2 -- G_31783693_RWE_Kraftwerk_Neurath/RConn2 -- 220_kV_Neurath_1a_CN_27919734_220000_CN31783693/LConn2
  380kV_Knechtsteden_West_CN_77179271_380000_CN31783693/RConn3 -- G_31783693_RWE_Kraftwerk_Neurath/RConn3 -- 220_kV_Neurath_1a_CN_27919734_220000_CN31783693/LConn3
  380kV_Knechtsteden_West_CN_77179271_380000_CN_207488608_380000/RConn1 -- T_207488608__/LConn1 -- 380_kV_Neurath_4d|5e_CN_207488608_380000_CN109373271/LConn1
  380kV_Knechtsteden_West_CN_77179271_380000_CN_207488608_380000/RConn2 -- T_207488608__/LConn2 -- 380_kV_Neurath_4d|5e_CN_207488608_380000_CN109373271/LConn2
  380kV_Knechtsteden_West_CN_77179271_380000_CN_207488608_380000/RConn3 -- T_207488608__/LConn3 -- 380_kV_Neurath_4d|5e_CN_207488608_380000_CN109373271/LConn3
  380kV_Meerbusch_West_CN_77179271_380000_CN_23380800_380000/RConn1 -- T_23380800_380000;220000;110000_Station_Utfort/LConn1 -- 380kV_Lohheide_West_CN_23380800_380000_CN26623135/RConn1
  380kV_Meerbusch_West_CN_77179271_380000_CN_23380800_380000/RConn2 -- T_23380800_380000;220000;110000_Station_Utfort/LConn2 -- 380kV_Lohheide_West_CN_23380800_380000_CN26623135/RConn2
  380kV_Meerbusch_West_CN_77179271_380000_CN_23380800_380000/RConn3 -- T_23380800_380000;220000;110000_Station_Utfort/LConn3 -- 380kV_Lohheide_West_CN_23380800_380000_CN26623135/RConn3
  T_25044557_380000_Station_Rath/LConn1 -- 380kV_Meerbusch_West_CN_77179271_380000_CN_25044557_380000/RConn1
  T_25044557_380000_Station_Rath/LConn2 -- 380kV_Meerbusch_West_CN_77179271_380000_CN_25044557_380000/RConn2
  T_25044557_380000_Station_Rath/LConn3 -- 380kV_Meerbusch_West_CN_77179271_380000_CN_25044557_380000/RConn3
  MP_CN_157806991_380000_CN178167136/LConn1 -- T_157806991_380000_Umspannwerk_Bärwalde/LConn1 -- 557_CN_157806991_380000_CN_157328339_380000/LConn1 -- 566_CN_157806991_380000_CN_30164703_380000/LConn1 -- 552_CN_157806991_380000_CN_157807291_380000/LConn1
  MP_CN_157806991_380000_CN178167136/LConn2 -- T_157806991_380000_Umspannwerk_Bärwalde/LConn2 -- 557_CN_157806991_380000_CN_157328339_380000/LConn2 -- 566_CN_157806991_380000_CN_30164703_380000/LConn2 -- 552_CN_157806991_380000_CN_157807291_380000/LConn2
  MP_CN_157806991_380000_CN178167136/LConn3 -- T_157806991_380000_Umspannwerk_Bärwalde/LConn3 -- 557_CN_157806991_380000_CN_157328339_380000/LConn3 -- 566_CN_157806991_380000_CN_30164703_380000/LConn3 -- 552_CN_157806991_380000_CN_157807291_380000/LConn3
  G_178167136_Kraftwerk_Boxberg/RConn1 -- MP_CN_157806991_380000_CN178167136/RConn1
  G_178167136_Kraftwerk_Boxberg/RConn2 -- MP_CN_157806991_380000_CN178167136/RConn2
  G_178167136_Kraftwerk_Boxberg/RConn3 -- MP_CN_157806991_380000_CN178167136/RConn3
  557_CN_157806991_380000_CN_157328339_380000/RConn1 -- T_157328339_380000;110000_Umspannwerk_Streumen/LConn1 -- 585_CN_157328339_380000_CN_32843531_380000/RConn1 -- 559_CN_157328339_380000_CN_23025610_380000/RConn1 -- 572_CN_23117075_380000_CN_157328339_380000/RConn1 -- 561_Streumen_CN_156683994_380000_CN_157328339_380000/RConn1
  557_CN_157806991_380000_CN_157328339_380000/RConn2 -- T_157328339_380000;110000_Umspannwerk_Streumen/LConn2 -- 585_CN_157328339_380000_CN_32843531_380000/RConn2 -- 559_CN_157328339_380000_CN_23025610_380000/RConn2 -- 572_CN_23117075_380000_CN_157328339_380000/RConn2 -- 561_Streumen_CN_156683994_380000_CN_157328339_380000/RConn2
  557_CN_157806991_380000_CN_157328339_380000/RConn3 -- T_157328339_380000;110000_Umspannwerk_Streumen/LConn3 -- 585_CN_157328339_380000_CN_32843531_380000/RConn3 -- 559_CN_157328339_380000_CN_23025610_380000/RConn3 -- 572_CN_23117075_380000_CN_157328339_380000/RConn3 -- 561_Streumen_CN_156683994_380000_CN_157328339_380000/RConn3
  566_CN_157806991_380000_CN_30164703_380000/RConn1 -- T_30164703_380000;110000_Graustein/LConn1 -- _CN_30164703_380000_CN58421134/LConn1 -- 561_CN_30164703_380000_CN_23025610_380000/RConn1
  566_CN_157806991_380000_CN_30164703_380000/RConn2 -- T_30164703_380000;110000_Graustein/LConn2 -- _CN_30164703_380000_CN58421134/LConn2 -- 561_CN_30164703_380000_CN_23025610_380000/RConn2
  566_CN_157806991_380000_CN_30164703_380000/RConn3 -- T_30164703_380000;110000_Graustein/LConn3 -- _CN_30164703_380000_CN58421134/LConn3 -- 561_CN_30164703_380000_CN_23025610_380000/RConn3
  552_CN_157806991_380000_CN_157807291_380000/RConn1 -- T_157807291_380000;110000_Umspannwerk_Schmölln/LConn1 -- Schmölln___Dresden_Süd___Röhrsdorf_CN_157807291_380000_CN_109917397_380000/LConn1 -- Schmölln___Dresden_Süd___Röhrsdorf_CN_157807291_380000_CN_23117075_380000/RConn1 -- Schmölln___Dresden_Süd___Röhrsdorf_CN_157807291_380000_CN_23241863_380000/LConn1 -- _CN_59026005_380000_CN_157807291_380000/LConn1
  552_CN_157806991_380000_CN_157807291_380000/RConn2 -- T_157807291_380000;110000_Umspannwerk_Schmölln/LConn2 -- Schmölln___Dresden_Süd___Röhrsdorf_CN_157807291_380000_CN_109917397_380000/LConn2 -- Schmölln___Dresden_Süd___Röhrsdorf_CN_157807291_380000_CN_23117075_380000/RConn2 -- Schmölln___Dresden_Süd___Röhrsdorf_CN_157807291_380000_CN_23241863_380000/LConn2 -- _CN_59026005_380000_CN_157807291_380000/LConn2
  552_CN_157806991_380000_CN_157807291_380000/RConn3 -- T_157807291_380000;110000_Umspannwerk_Schmölln/LConn3 -- Schmölln___Dresden_Süd___Röhrsdorf_CN_157807291_380000_CN_109917397_380000/LConn3 -- Schmölln___Dresden_Süd___Röhrsdorf_CN_157807291_380000_CN_23117075_380000/RConn3 -- Schmölln___Dresden_Süd___Röhrsdorf_CN_157807291_380000_CN_23241863_380000/LConn3 -- _CN_59026005_380000_CN_157807291_380000/LConn3
  305_CN_35176751_380000_CN_301158539_380000/LConn1 -- T_35176751_380000;110000_Audorf/LConn1 -- 305_CN_35176751_380000_CN_87952821_380000/LConn1 -- 303_CN_35176751_380000_CN_28502915_380000/RConn1
  305_CN_35176751_380000_CN_301158539_380000/LConn2 -- T_35176751_380000;110000_Audorf/LConn2 -- 305_CN_35176751_380000_CN_87952821_380000/LConn2 -- 303_CN_35176751_380000_CN_28502915_380000/RConn2
  305_CN_35176751_380000_CN_301158539_380000/LConn3 -- T_35176751_380000;110000_Audorf/LConn3 -- 305_CN_35176751_380000_CN_87952821_380000/LConn3 -- 303_CN_35176751_380000_CN_28502915_380000/RConn3
  T_301158539_380000;110000;20000_Umspannwerk_Jardelund/LConn1 -- 305_CN_35176751_380000_CN_301158539_380000/RConn1
  T_301158539_380000;110000;20000_Umspannwerk_Jardelund/LConn2 -- 305_CN_35176751_380000_CN_301158539_380000/RConn2
  T_301158539_380000;110000;20000_Umspannwerk_Jardelund/LConn3 -- 305_CN_35176751_380000_CN_301158539_380000/RConn3
  T_87952821_380000;220000;110000;20000_Flensburg/LConn1 -- 305_CN_35176751_380000_CN_87952821_380000/RConn1
  T_87952821_380000;220000;110000;20000_Flensburg/LConn2 -- 305_CN_35176751_380000_CN_87952821_380000/RConn2
  T_87952821_380000;220000;110000;20000_Flensburg/LConn3 -- 305_CN_35176751_380000_CN_87952821_380000/RConn3
  T_159326655_220000;110000_Obrigheim/LConn1 -- _CN_25557397_220000_CN_159326655_220000/RConn1
  T_159326655_220000;110000_Obrigheim/LConn2 -- _CN_25557397_220000_CN_159326655_220000/RConn2
  T_159326655_220000;110000_Obrigheim/LConn3 -- _CN_25557397_220000_CN_159326655_220000/RConn3
  T_42050342_380000;220000;110000_Umspannwerk_Goldshöfe/RConn1 -- _CN_25557397_220000_CN_42050342_220000/RConn1
  T_42050342_380000;220000;110000_Umspannwerk_Goldshöfe/RConn2 -- _CN_25557397_220000_CN_42050342_220000/RConn2
  T_42050342_380000;220000;110000_Umspannwerk_Goldshöfe/RConn3 -- _CN_25557397_220000_CN_42050342_220000/RConn3
  T_104878489_220000;110000_Umspannwerk_Kraftwerk_Emden/LConn1 -- _CN_104878489_220000_CN_34835258_220000/LConn1
  T_104878489_220000;110000_Umspannwerk_Kraftwerk_Emden/LConn2 -- _CN_104878489_220000_CN_34835258_220000/LConn2
  T_104878489_220000;110000_Umspannwerk_Kraftwerk_Emden/LConn3 -- _CN_104878489_220000_CN_34835258_220000/LConn3
  _CN_104878489_220000_CN_34835258_220000/RConn1 -- T_34835258_220000;110000_Emden_Borßum/LConn1 -- 203_CN_34835258_220000_CN_173178563_220000/LConn1
  _CN_104878489_220000_CN_34835258_220000/RConn2 -- T_34835258_220000;110000_Emden_Borßum/LConn2 -- 203_CN_34835258_220000_CN_173178563_220000/LConn2
  _CN_104878489_220000_CN_34835258_220000/RConn3 -- T_34835258_220000;110000_Emden_Borßum/LConn3 -- 203_CN_34835258_220000_CN_173178563_220000/LConn3
  T_143882655_380000;220000;110000_Umspannwerk_Vieselbach/RConn1 -- Wolkramshausen_CN_143882655_220000_CN_157164284_220000/LConn1
  T_143882655_380000;220000;110000_Umspannwerk_Vieselbach/RConn2 -- Wolkramshausen_CN_143882655_220000_CN_157164284_220000/LConn2
  T_143882655_380000;220000;110000_Umspannwerk_Vieselbach/RConn3 -- Wolkramshausen_CN_143882655_220000_CN_157164284_220000/LConn3
  Wolkramshausen_CN_143882655_220000_CN_157164284_220000/RConn1 -- T_157164284_220000_Wolkramshausen_(220_kV)/LConn1 -- 358_CN_157164284_220000_CN_22879599_220000/LConn1
  Wolkramshausen_CN_143882655_220000_CN_157164284_220000/RConn2 -- T_157164284_220000_Wolkramshausen_(220_kV)/LConn2 -- 358_CN_157164284_220000_CN_22879599_220000/LConn2
  Wolkramshausen_CN_143882655_220000_CN_157164284_220000/RConn3 -- T_157164284_220000_Wolkramshausen_(220_kV)/LConn3 -- 358_CN_157164284_220000_CN_22879599_220000/LConn3
  _CN_143882655_380000_CN_29309786_380000/RConn1 -- T_29309786_380000;110000_Mecklar/LConn1 -- _CN_29309786_380000_CN_156673636_380000/LConn1 -- _CN_29309786_380000_CN_148446247_380000/LConn1
  _CN_143882655_380000_CN_29309786_380000/RConn2 -- T_29309786_380000;110000_Mecklar/LConn2 -- _CN_29309786_380000_CN_156673636_380000/LConn2 -- _CN_29309786_380000_CN_148446247_380000/LConn2
  _CN_143882655_380000_CN_29309786_380000/RConn3 -- T_29309786_380000;110000_Mecklar/LConn3 -- _CN_29309786_380000_CN_156673636_380000/LConn3 -- _CN_29309786_380000_CN_148446247_380000/LConn3
  T_154418450_380000;110000_Eisenach/LConn1 -- _CN_143882655_380000_CN_154418450_380000/RConn1
  T_154418450_380000;110000_Eisenach/LConn2 -- _CN_143882655_380000_CN_154418450_380000/RConn2
  T_154418450_380000;110000_Eisenach/LConn3 -- _CN_143882655_380000_CN_154418450_380000/RConn3
  T_148211527_380000;110000_Großschwabhausen/LConn1 -- _CN_143882655_380000_CN_148211527_380000/RConn1
  T_148211527_380000;110000_Großschwabhausen/LConn2 -- _CN_143882655_380000_CN_148211527_380000/RConn2
  T_148211527_380000;110000_Großschwabhausen/LConn3 -- _CN_143882655_380000_CN_148211527_380000/RConn3
  _CN_145486242_220000_CN145861680/LConn1 -- T_145486242__/LConn1 -- _CN_145486242_220000_CN_42410916_220000/LConn1
  _CN_145486242_220000_CN145861680/LConn2 -- T_145486242__/LConn2 -- _CN_145486242_220000_CN_42410916_220000/LConn2
  _CN_145486242_220000_CN145861680/LConn3 -- T_145486242__/LConn3 -- _CN_145486242_220000_CN_42410916_220000/LConn3
  _CN_145486242_220000_CN145861680/RConn1 -- G_145861680_Kraftwerk_Staudinger/RConn1 -- _CN_23881272_220000_CN145861680/LConn1 -- _CN_42411962_220000_CN145861680/LConn1 -- 2205;III;IIII_CN_55069713_220000_CN145861680/LConn1 -- _CN_42410916_220000_CN145861680/LConn1
  _CN_145486242_220000_CN145861680/RConn2 -- G_145861680_Kraftwerk_Staudinger/RConn2 -- _CN_23881272_220000_CN145861680/LConn2 -- _CN_42411962_220000_CN145861680/LConn2 -- 2205;III;IIII_CN_55069713_220000_CN145861680/LConn2 -- _CN_42410916_220000_CN145861680/LConn2
  _CN_145486242_220000_CN145861680/RConn3 -- G_145861680_Kraftwerk_Staudinger/RConn3 -- _CN_23881272_220000_CN145861680/LConn3 -- _CN_42411962_220000_CN145861680/LConn3 -- 2205;III;IIII_CN_55069713_220000_CN145861680/LConn3 -- _CN_42410916_220000_CN145861680/LConn3
  _CN_145486242_220000_CN_42410916_220000/RConn1 -- T_42410916_380000;220000_Umspannwerk_Großkrotzenburg/RConn1 -- _CN_42410916_220000_CN145861680/RConn1 -- _CN_42410916_220000_CN_193674783_220000/LConn1 -- L_42410916/LConn1
  _CN_145486242_220000_CN_42410916_220000/RConn2 -- T_42410916_380000;220000_Umspannwerk_Großkrotzenburg/RConn2 -- _CN_42410916_220000_CN145861680/RConn2 -- _CN_42410916_220000_CN_193674783_220000/LConn2 -- L_42410916/LConn2
  _CN_145486242_220000_CN_42410916_220000/RConn3 -- T_42410916_380000;220000_Umspannwerk_Großkrotzenburg/RConn3 -- _CN_42410916_220000_CN145861680/RConn3 -- _CN_42410916_220000_CN_193674783_220000/LConn3 -- L_42410916/LConn3
  T_24267175_220000;110000_Umspannanlage_Frimmersdorf_I/LConn1 -- _CN_24267175_220000_CN24267119/LConn1
  T_24267175_220000;110000_Umspannanlage_Frimmersdorf_I/LConn2 -- _CN_24267175_220000_CN24267119/LConn2
  T_24267175_220000;110000_Umspannanlage_Frimmersdorf_I/LConn3 -- _CN_24267175_220000_CN24267119/LConn3
  _CN_24267175_220000_CN24267119/RConn1 -- G_24267119_RWE_Kraftwerk_Frimmersdorf/RConn1 -- 220_kV_Neurath_1a_CN_27919734_220000_CN24267119/LConn1
  _CN_24267175_220000_CN24267119/RConn2 -- G_24267119_RWE_Kraftwerk_Frimmersdorf/RConn2 -- 220_kV_Neurath_1a_CN_27919734_220000_CN24267119/LConn2
  _CN_24267175_220000_CN24267119/RConn3 -- G_24267119_RWE_Kraftwerk_Frimmersdorf/RConn3 -- 220_kV_Neurath_1a_CN_27919734_220000_CN24267119/LConn3
  T_151507370_220000_/LConn1 -- _CN_151507370_220000_CN_28227099_220000/RConn1
  T_151507370_220000_/LConn2 -- _CN_151507370_220000_CN_28227099_220000/RConn2
  T_151507370_220000_/LConn3 -- _CN_151507370_220000_CN_28227099_220000/RConn3
  T_50643382_220000_Cloppenburg_220_kV/LConn1 -- 206_CN_50643382_220000_CN_173178563_220000/LConn1
  T_50643382_220000_Cloppenburg_220_kV/LConn2 -- 206_CN_50643382_220000_CN_173178563_220000/LConn2
  T_50643382_220000_Cloppenburg_220_kV/LConn3 -- 206_CN_50643382_220000_CN_173178563_220000/LConn3
  206_CN_50643382_220000_CN_173178563_220000/RConn1 -- T_173178563_220000;110000_Conneforde_110_220_kV/LConn1 -- 302_CN_32076853_220000_CN_173178563_220000/LConn1 -- 204_CN_173178563_220000_CN_23744346_220000/LConn1 -- 203_CN_34835258_220000_CN_173178563_220000/RConn1 -- Conneforde_220_kV_CN_23837631_220000_CN_173178563_220000/LConn1
  206_CN_50643382_220000_CN_173178563_220000/RConn2 -- T_173178563_220000;110000_Conneforde_110_220_kV/LConn2 -- 302_CN_32076853_220000_CN_173178563_220000/LConn2 -- 204_CN_173178563_220000_CN_23744346_220000/LConn2 -- 203_CN_34835258_220000_CN_173178563_220000/RConn2 -- Conneforde_220_kV_CN_23837631_220000_CN_173178563_220000/LConn2
  206_CN_50643382_220000_CN_173178563_220000/RConn3 -- T_173178563_220000;110000_Conneforde_110_220_kV/LConn3 -- 302_CN_32076853_220000_CN_173178563_220000/LConn3 -- 204_CN_173178563_220000_CN_23744346_220000/LConn3 -- 203_CN_34835258_220000_CN_173178563_220000/RConn3 -- Conneforde_220_kV_CN_23837631_220000_CN_173178563_220000/LConn3
  T_68532663_220000;110000_Umspannwerk_Krün/LConn1 -- _CN_68532663_220000_CN_24237879_220000/LConn1
  T_68532663_220000;110000_Umspannwerk_Krün/LConn2 -- _CN_68532663_220000_CN_24237879_220000/LConn2
  T_68532663_220000;110000_Umspannwerk_Krün/LConn3 -- _CN_68532663_220000_CN_24237879_220000/LConn3
  _CN_68532663_220000_CN_24237879_220000/RConn1 -- T_24237879_220000;110000_Umspannwerk_Oberbrunn/LConn1 -- Oberbrunn___Oberbachern_CN_18629425_220000_CN_24237879_220000/LConn1
  _CN_68532663_220000_CN_24237879_220000/RConn2 -- T_24237879_220000;110000_Umspannwerk_Oberbrunn/LConn2 -- Oberbrunn___Oberbachern_CN_18629425_220000_CN_24237879_220000/LConn2
  _CN_68532663_220000_CN_24237879_220000/RConn3 -- T_24237879_220000;110000_Umspannwerk_Oberbrunn/LConn3 -- Oberbrunn___Oberbachern_CN_18629425_220000_CN_24237879_220000/LConn3
  T_26383042_380000;220000;110000;10000_Umspannwerk_Blankenhagen/RConn1 -- _CN_37764852_220000_CN_26383042_220000/RConn1
  T_26383042_380000;220000;110000;10000_Umspannwerk_Blankenhagen/RConn2 -- _CN_37764852_220000_CN_26383042_220000/RConn2
  T_26383042_380000;220000;110000;10000_Umspannwerk_Blankenhagen/RConn3 -- _CN_37764852_220000_CN_26383042_220000/RConn3
  T_39229429_220000;110000_Station_Hesseln/LConn1 -- _CN_37764852_220000_CN_39229429_220000/RConn1
  T_39229429_220000;110000_Station_Hesseln/LConn2 -- _CN_37764852_220000_CN_39229429_220000/RConn2
  T_39229429_220000;110000_Station_Hesseln/LConn3 -- _CN_37764852_220000_CN_39229429_220000/RConn3
  T_32993727_220000;110000_KW_Niederaußem/LConn1 -- 220_kV_Niederaußem_3c_CN_32993727_220000_CN-1726424/RConn1
  T_32993727_220000;110000_KW_Niederaußem/LConn2 -- 220_kV_Niederaußem_3c_CN_32993727_220000_CN-1726424/RConn2
  T_32993727_220000;110000_KW_Niederaußem/LConn3 -- 220_kV_Niederaußem_3c_CN_32993727_220000_CN-1726424/RConn3
  Oberbachern___Neufinsing_CN_24158385_220000_CN_18629425_220000/RConn1 -- T_18629425_380000;220000;110000_Umspannwerk_Oberbachern/RConn1 -- Oberbrunn___Oberbachern_CN_18629425_220000_CN_24237879_220000/RConn1
  Oberbachern___Neufinsing_CN_24158385_220000_CN_18629425_220000/RConn2 -- T_18629425_380000;220000;110000_Umspannwerk_Oberbachern/RConn2 -- Oberbrunn___Oberbachern_CN_18629425_220000_CN_24237879_220000/RConn2
  Oberbachern___Neufinsing_CN_24158385_220000_CN_18629425_220000/RConn3 -- T_18629425_380000;220000;110000_Umspannwerk_Oberbachern/RConn3 -- Oberbrunn___Oberbachern_CN_18629425_220000_CN_24237879_220000/RConn3
  Neufinsing___Zolling_CN_24158385_220000_CN_133342285_220000/RConn1 -- T_133342285_220000;110000_Zolling___Irsching/LConn1 -- _CN_232833796_220000_CN_133342285_220000/LConn1
  Neufinsing___Zolling_CN_24158385_220000_CN_133342285_220000/RConn2 -- T_133342285_220000;110000_Zolling___Irsching/LConn2 -- _CN_232833796_220000_CN_133342285_220000/LConn2
  Neufinsing___Zolling_CN_24158385_220000_CN_133342285_220000/RConn3 -- T_133342285_220000;110000_Zolling___Irsching/LConn3 -- _CN_232833796_220000_CN_133342285_220000/LConn3
  Neufinsing___Zolling_CN_24158385_220000_CN_137602559_220000/RConn1 -- T_137602559_380000;220000;110000_Irsching/RConn1 -- _CN_137602559_220000_CN29122363/LConn1
  Neufinsing___Zolling_CN_24158385_220000_CN_137602559_220000/RConn2 -- T_137602559_380000;220000;110000_Irsching/RConn2 -- _CN_137602559_220000_CN29122363/LConn2
  Neufinsing___Zolling_CN_24158385_220000_CN_137602559_220000/RConn3 -- T_137602559_380000;220000;110000_Irsching/RConn3 -- _CN_137602559_220000_CN29122363/LConn3
  T_75865676_220000_Umspannwerk_Marienberg/LConn1 -- _CN_24158385_220000_CN_75865676_220000/RConn1
  T_75865676_220000_Umspannwerk_Marienberg/LConn2 -- _CN_24158385_220000_CN_75865676_220000/RConn2
  T_75865676_220000_Umspannwerk_Marienberg/LConn3 -- _CN_24158385_220000_CN_75865676_220000/RConn3
  _CN_35833592_220000_CN_35833442_220000/RConn1 -- T_35833442_220000_/LConn1 -- _CN_35833442_220000_CN125808869/LConn1
  _CN_35833592_220000_CN_35833442_220000/RConn2 -- T_35833442_220000_/LConn2 -- _CN_35833442_220000_CN125808869/LConn2
  _CN_35833592_220000_CN_35833442_220000/RConn3 -- T_35833442_220000_/LConn3 -- _CN_35833442_220000_CN125808869/LConn3
  T_158253525_220000;110000_Umspannwerk_Paderborn_Süd/LConn1 -- _CN_158253525_220000_CN_24264701_220000/RConn1
  T_158253525_220000;110000_Umspannwerk_Paderborn_Süd/LConn2 -- _CN_158253525_220000_CN_24264701_220000/RConn2
  T_158253525_220000;110000_Umspannwerk_Paderborn_Süd/LConn3 -- _CN_158253525_220000_CN_24264701_220000/RConn3
  493_CN_26472665_380000_CN_30132758_380000/RConn1 -- T_30132758_380000;110000_Teufelsbruch/LConn1 -- _CN_30132758_380000_CN185569568/LConn1
  493_CN_26472665_380000_CN_30132758_380000/RConn2 -- T_30132758_380000;110000_Teufelsbruch/LConn2 -- _CN_30132758_380000_CN185569568/LConn2
  493_CN_26472665_380000_CN_30132758_380000/RConn3 -- T_30132758_380000;110000_Teufelsbruch/LConn3 -- _CN_30132758_380000_CN185569568/LConn3
  T_32690742_380000;110000_Umspannwerk_Klostermansfeld/LConn1 -- 536_CN_26472665_380000_CN_32690742_380000/RConn1
  T_32690742_380000;110000_Umspannwerk_Klostermansfeld/LConn2 -- 536_CN_26472665_380000_CN_32690742_380000/RConn2
  T_32690742_380000;110000_Umspannwerk_Klostermansfeld/LConn3 -- 536_CN_26472665_380000_CN_32690742_380000/RConn3
  _CN_24414688_220000_CN_42507488_220000/RConn1 -- T_24414688_220000;110000_Station_Wambel/LConn1 -- _CN_24414688_220000_CN_24858617_220000/LConn1
  _CN_24414688_220000_CN_42507488_220000/RConn2 -- T_24414688_220000;110000_Station_Wambel/LConn2 -- _CN_24414688_220000_CN_24858617_220000/LConn2
  _CN_24414688_220000_CN_42507488_220000/RConn3 -- T_24414688_220000;110000_Station_Wambel/LConn3 -- _CN_24414688_220000_CN_24858617_220000/LConn3
  T_24858617_220000_Ratsbusch/LConn1 -- _CN_24414688_220000_CN_24858617_220000/RConn1
  T_24858617_220000_Ratsbusch/LConn2 -- _CN_24414688_220000_CN_24858617_220000/RConn2
  T_24858617_220000_Ratsbusch/LConn3 -- _CN_24414688_220000_CN_24858617_220000/RConn3
  Meitingen_Nord;_Süd_CN_24652261_380000_CN_88945213_380000/RConn1 -- T_88945213_380000_Umspannwerk_Gundelfingen/LConn1 -- _CN_88945213_380000_CN31023006/LConn1 -- _CN_88945213_380000_CN_31019939_380000/LConn1
  Meitingen_Nord;_Süd_CN_24652261_380000_CN_88945213_380000/RConn2 -- T_88945213_380000_Umspannwerk_Gundelfingen/LConn2 -- _CN_88945213_380000_CN31023006/LConn2 -- _CN_88945213_380000_CN_31019939_380000/LConn2
  Meitingen_Nord;_Süd_CN_24652261_380000_CN_88945213_380000/RConn3 -- T_88945213_380000_Umspannwerk_Gundelfingen/LConn3 -- _CN_88945213_380000_CN31023006/LConn3 -- _CN_88945213_380000_CN_31019939_380000/LConn3
  T_76246159_380000;110000_Umspannwerk_Meitingen/LConn1 -- _CN_24652261_380000_CN_76246159_380000/RConn1
  T_76246159_380000;110000_Umspannwerk_Meitingen/LConn2 -- _CN_24652261_380000_CN_76246159_380000/RConn2
  T_76246159_380000;110000_Umspannwerk_Meitingen/LConn3 -- _CN_24652261_380000_CN_76246159_380000/RConn3
  358_CN_157164284_220000_CN_22879599_220000/RConn1 -- T_22879599_220000;110000_Umspannwerk_Großdalzig/LConn1 -- _CN_22879599_220000_CN_32843531_220000/LConn1
  358_CN_157164284_220000_CN_22879599_220000/RConn2 -- T_22879599_220000;110000_Umspannwerk_Großdalzig/LConn2 -- _CN_22879599_220000_CN_32843531_220000/LConn2
  358_CN_157164284_220000_CN_22879599_220000/RConn3 -- T_22879599_220000;110000_Umspannwerk_Großdalzig/LConn3 -- _CN_22879599_220000_CN_32843531_220000/LConn3
  T_229500139_220000_DOW/LConn1 -- _CN_151765495_220000_CN_229500139_220000/RConn1
  T_229500139_220000_DOW/LConn2 -- _CN_151765495_220000_CN_229500139_220000/RConn2
  T_229500139_220000_DOW/LConn3 -- _CN_151765495_220000_CN_229500139_220000/RConn3
  419_Krümmel___Görries_CN_30040568_380000_CN_23366603_380000/LConn1 -- T_30040568_380000;110000_Görries/LConn1 -- 419_Krümmel___Görries_CN_30040568_380000_CN_234171369_380000/LConn1 -- 419_Krümmel___Görries_CN_30040568_380000_CN_32062544_380000/RConn1
  419_Krümmel___Görries_CN_30040568_380000_CN_23366603_380000/LConn2 -- T_30040568_380000;110000_Görries/LConn2 -- 419_Krümmel___Görries_CN_30040568_380000_CN_234171369_380000/LConn2 -- 419_Krümmel___Görries_CN_30040568_380000_CN_32062544_380000/RConn2
  419_Krümmel___Görries_CN_30040568_380000_CN_23366603_380000/LConn3 -- T_30040568_380000;110000_Görries/LConn3 -- 419_Krümmel___Görries_CN_30040568_380000_CN_234171369_380000/LConn3 -- 419_Krümmel___Görries_CN_30040568_380000_CN_32062544_380000/RConn3
  419_Krümmel___Görries_CN_30040568_380000_CN_23366603_380000/RConn1 -- T_23366603_380000;110000_Krümmel/LConn1 -- KKW_Krümmel___UW_HH_OST_CN_23366603_380000_CN_23583867_380000/RConn1 -- _CN_23366603_380000_CN_28327356_380000/LConn1
  419_Krümmel___Görries_CN_30040568_380000_CN_23366603_380000/RConn2 -- T_23366603_380000;110000_Krümmel/LConn2 -- KKW_Krümmel___UW_HH_OST_CN_23366603_380000_CN_23583867_380000/RConn2 -- _CN_23366603_380000_CN_28327356_380000/LConn2
  419_Krümmel___Görries_CN_30040568_380000_CN_23366603_380000/RConn3 -- T_23366603_380000;110000_Krümmel/LConn3 -- KKW_Krümmel___UW_HH_OST_CN_23366603_380000_CN_23583867_380000/RConn3 -- _CN_23366603_380000_CN_28327356_380000/LConn3
  T_234171369_380000_Wessin/LConn1 -- 419_Krümmel___Görries_CN_30040568_380000_CN_234171369_380000/RConn1
  T_234171369_380000_Wessin/LConn2 -- 419_Krümmel___Görries_CN_30040568_380000_CN_234171369_380000/RConn2
  T_234171369_380000_Wessin/LConn3 -- 419_Krümmel___Görries_CN_30040568_380000_CN_234171369_380000/RConn3
  380kV_Twistetal_Ost_3_CN_42797575_380000_CN_41232144_380000/RConn1 -- T_41232144_380000;110000_Umspannwerk_Twistetal/LConn1 -- Leitung_3212;Leitung_3213_CN_156673636_380000_CN_41232144_380000/LConn1
  380kV_Twistetal_Ost_3_CN_42797575_380000_CN_41232144_380000/RConn2 -- T_41232144_380000;110000_Umspannwerk_Twistetal/LConn2 -- Leitung_3212;Leitung_3213_CN_156673636_380000_CN_41232144_380000/LConn2
  380kV_Twistetal_Ost_3_CN_42797575_380000_CN_41232144_380000/RConn3 -- T_41232144_380000;110000_Umspannwerk_Twistetal/LConn3 -- Leitung_3212;Leitung_3213_CN_156673636_380000_CN_41232144_380000/LConn3
  380kV_Twistetal_Ost_3_CN_42797575_380000_CN_25943440_380000/RConn1 -- T_25943440_380000;110000_Umspannwerk_Elsen/LConn1 -- _CN_25943440_380000_CN_24264701_380000/LConn1
  380kV_Twistetal_Ost_3_CN_42797575_380000_CN_25943440_380000/RConn2 -- T_25943440_380000;110000_Umspannwerk_Elsen/LConn2 -- _CN_25943440_380000_CN_24264701_380000/LConn2
  380kV_Twistetal_Ost_3_CN_42797575_380000_CN_25943440_380000/RConn3 -- T_25943440_380000;110000_Umspannwerk_Elsen/LConn3 -- _CN_25943440_380000_CN_24264701_380000/LConn3
  _CN_152261133_220000_CN_163093653_220000/RConn1 -- T_163093653_220000;110000_Mannheim/LConn1 -- _CN_163093653_220000_CN152506744/RConn1
  _CN_152261133_220000_CN_163093653_220000/RConn2 -- T_163093653_220000;110000_Mannheim/LConn2 -- _CN_163093653_220000_CN152506744/RConn2
  _CN_152261133_220000_CN_163093653_220000/RConn3 -- T_163093653_220000;110000_Mannheim/LConn3 -- _CN_163093653_220000_CN152506744/RConn3
  T_160929097_220000;110000_Umspannwerk_Weinheim/LConn1 -- _CN_152261133_220000_CN_160929097_220000/RConn1
  T_160929097_220000;110000_Umspannwerk_Weinheim/LConn2 -- _CN_152261133_220000_CN_160929097_220000/RConn2
  T_160929097_220000;110000_Umspannwerk_Weinheim/LConn3 -- _CN_152261133_220000_CN_160929097_220000/RConn3
  T_154729020_220000;110000_Umspannwerk_Altlußheim/LConn1 -- _CN_152261133_220000_CN_154729020_220000/RConn1
  T_154729020_220000;110000_Umspannwerk_Altlußheim/LConn2 -- _CN_152261133_220000_CN_154729020_220000/RConn2
  T_154729020_220000;110000_Umspannwerk_Altlußheim/LConn3 -- _CN_152261133_220000_CN_154729020_220000/RConn3
  _CN_152261133_380000_CN_149987048_380000/RConn1 -- T_149987048_380000;220000_Station_Bürstadt/LConn1 -- 2_x_380_kV;_3_x_220_kV_CN_23284340_380000_CN_149987048_380000/LConn1 -- _CN_160584794_380000_CN_149987048_380000/LConn1 -- _CN_25802269_380000_CN_149987048_380000/LConn1
  _CN_152261133_380000_CN_149987048_380000/RConn2 -- T_149987048_380000;220000_Station_Bürstadt/LConn2 -- 2_x_380_kV;_3_x_220_kV_CN_23284340_380000_CN_149987048_380000/LConn2 -- _CN_160584794_380000_CN_149987048_380000/LConn2 -- _CN_25802269_380000_CN_149987048_380000/LConn2
  _CN_152261133_380000_CN_149987048_380000/RConn3 -- T_149987048_380000;220000_Station_Bürstadt/LConn3 -- 2_x_380_kV;_3_x_220_kV_CN_23284340_380000_CN_149987048_380000/LConn3 -- _CN_160584794_380000_CN_149987048_380000/LConn3 -- _CN_25802269_380000_CN_149987048_380000/LConn3
  _CN_152261133_380000_CN_152018146_380000/RConn1 -- T_152018146_380000_Mittelbexbach/LConn1 -- _CN_152018146_380000_CN28051874/RConn1
  _CN_152261133_380000_CN_152018146_380000/RConn2 -- T_152018146_380000_Mittelbexbach/LConn2 -- _CN_152018146_380000_CN28051874/RConn2
  _CN_152261133_380000_CN_152018146_380000/RConn3 -- T_152018146_380000_Mittelbexbach/LConn3 -- _CN_152018146_380000_CN28051874/RConn3
  7563_CN_152261133_380000_CN152261126/RConn1 -- G_152261126_Rheinhafen_Dampfkraftwerk/RConn1 -- 7563_CN_272646943_380000_CN152261126/LConn1 -- 7564_CN_194446360_380000_CN152261126/LConn1
  7563_CN_152261133_380000_CN152261126/RConn2 -- G_152261126_Rheinhafen_Dampfkraftwerk/RConn2 -- 7563_CN_272646943_380000_CN152261126/LConn2 -- 7564_CN_194446360_380000_CN152261126/LConn2
  7563_CN_152261133_380000_CN152261126/RConn3 -- G_152261126_Rheinhafen_Dampfkraftwerk/RConn3 -- 7563_CN_272646943_380000_CN152261126/LConn3 -- 7564_CN_194446360_380000_CN152261126/LConn3
  T_32966636_220000;110000_220_kV_Umspannwerk_Birkenfeld/LConn1 -- _CN_152261133_220000_CN_32966636_220000/RConn1
  T_32966636_220000;110000_220_kV_Umspannwerk_Birkenfeld/LConn2 -- _CN_152261133_220000_CN_32966636_220000/RConn2
  T_32966636_220000;110000_220_kV_Umspannwerk_Birkenfeld/LConn3 -- _CN_152261133_220000_CN_32966636_220000/RConn3
  _CN_152261133_220000_CN_32725957_220000/RConn1 -- T_32725957_220000;110000_Umspannwerk_Oberwald/LConn1 -- _CN_32725957_220000_CN_32725958_220000/LConn1
  _CN_152261133_220000_CN_32725957_220000/RConn2 -- T_32725957_220000;110000_Umspannwerk_Oberwald/LConn2 -- _CN_32725957_220000_CN_32725958_220000/LConn2
  _CN_152261133_220000_CN_32725957_220000/RConn3 -- T_32725957_220000;110000_Umspannwerk_Oberwald/LConn3 -- _CN_32725957_220000_CN_32725958_220000/LConn3
  T_242756113_380000;220000;110000_380_kV_Umspannwerk_Eichstetten/RConn1 -- _CN_242756113_220000_CN_87653464_220000/LConn1
  T_242756113_380000;220000;110000_380_kV_Umspannwerk_Eichstetten/RConn2 -- _CN_242756113_220000_CN_87653464_220000/LConn2
  T_242756113_380000;220000;110000_380_kV_Umspannwerk_Eichstetten/RConn3 -- _CN_242756113_220000_CN_87653464_220000/LConn3
  _CN_242756113_220000_CN_87653464_220000/RConn1 -- T_87653464_220000;110000_220_kV_Umspannwerk_Eichstetten/LConn1 -- _CN_31367937_220000_CN_87653464_220000/LConn1 -- _CN_87653464_220000_CN_146962222_220000/RConn1
  _CN_242756113_220000_CN_87653464_220000/RConn2 -- T_87653464_220000;110000_220_kV_Umspannwerk_Eichstetten/LConn2 -- _CN_31367937_220000_CN_87653464_220000/LConn2 -- _CN_87653464_220000_CN_146962222_220000/RConn2
  _CN_242756113_220000_CN_87653464_220000/RConn3 -- T_87653464_220000;110000_220_kV_Umspannwerk_Eichstetten/LConn3 -- _CN_31367937_220000_CN_87653464_220000/LConn3 -- _CN_87653464_220000_CN_146962222_220000/RConn3
  380kV_Lippe_Süd_CN_23022100_380000_CN_24462426_380000/RConn1 -- T_24462426_380000;220000;110000_Station_Niederrhein/LConn1 -- _CN_24462426_380000_CN401873466/LConn1
  380kV_Lippe_Süd_CN_23022100_380000_CN_24462426_380000/RConn2 -- T_24462426_380000;220000;110000_Station_Niederrhein/LConn2 -- _CN_24462426_380000_CN401873466/LConn2
  380kV_Lippe_Süd_CN_23022100_380000_CN_24462426_380000/RConn3 -- T_24462426_380000;220000;110000_Station_Niederrhein/LConn3 -- _CN_24462426_380000_CN401873466/LConn3
  T_24280460_380000;110000_Station_Nordlicht/LConn1 -- 380kV_Kusenhorst_CN_23022100_380000_CN_24280460_380000/RConn1
  T_24280460_380000;110000_Station_Nordlicht/LConn2 -- 380kV_Kusenhorst_CN_23022100_380000_CN_24280460_380000/RConn2
  T_24280460_380000;110000_Station_Nordlicht/LConn3 -- 380kV_Kusenhorst_CN_23022100_380000_CN_24280460_380000/RConn3
  T_26291794_380000;110000_Station_Rosenblumendelle/LConn1 -- 380kV_Kusenhorst_CN_23022100_380000_CN_26291794_380000/RConn1
  T_26291794_380000;110000_Station_Rosenblumendelle/LConn2 -- 380kV_Kusenhorst_CN_23022100_380000_CN_26291794_380000/RConn2
  T_26291794_380000;110000_Station_Rosenblumendelle/LConn3 -- 380kV_Kusenhorst_CN_23022100_380000_CN_26291794_380000/RConn3
  T_24921206_380000;220000_Station_Büscherhof/LConn1 -- 380kV_Kusenhorst_CN_23022100_380000_CN_24921206_380000/RConn1
  T_24921206_380000;220000_Station_Büscherhof/LConn2 -- 380kV_Kusenhorst_CN_23022100_380000_CN_24921206_380000/RConn2
  T_24921206_380000;220000_Station_Büscherhof/LConn3 -- 380kV_Kusenhorst_CN_23022100_380000_CN_24921206_380000/RConn3
  _CN_30132758_380000_CN185569568/RConn1 -- G_185569568_Heizkraftwerk_Reuter_West/RConn1 -- 903;_904_CN_11500045_380000_CN185569568/LConn1 -- _CN_43163132_380000_CN185569568/LConn1
  _CN_30132758_380000_CN185569568/RConn2 -- G_185569568_Heizkraftwerk_Reuter_West/RConn2 -- 903;_904_CN_11500045_380000_CN185569568/LConn2 -- _CN_43163132_380000_CN185569568/LConn2
  _CN_30132758_380000_CN185569568/RConn3 -- G_185569568_Heizkraftwerk_Reuter_West/RConn3 -- 903;_904_CN_11500045_380000_CN185569568/LConn3 -- _CN_43163132_380000_CN185569568/LConn3
  T_78441561_380000;110000_Umspannwerk_Plattling/LConn1 -- Pleinting___Plattling___Schwandorf_CN_78441561_380000_CN_28956649_380000/LConn1
  T_78441561_380000;110000_Umspannwerk_Plattling/LConn2 -- Pleinting___Plattling___Schwandorf_CN_78441561_380000_CN_28956649_380000/LConn2
  T_78441561_380000;110000_Umspannwerk_Plattling/LConn3 -- Pleinting___Plattling___Schwandorf_CN_78441561_380000_CN_28956649_380000/LConn3
  Pleinting___Plattling___Schwandorf_CN_78441561_380000_CN_28956649_380000/RConn1 -- T_28956649_380000;220000;110000_Schwandorf/LConn1 -- Schwandorf___Etzenricht_CN_29084374_380000_CN_28956649_380000/RConn1
  Pleinting___Plattling___Schwandorf_CN_78441561_380000_CN_28956649_380000/RConn2 -- T_28956649_380000;220000;110000_Schwandorf/LConn2 -- Schwandorf___Etzenricht_CN_29084374_380000_CN_28956649_380000/RConn2
  Pleinting___Plattling___Schwandorf_CN_78441561_380000_CN_28956649_380000/RConn3 -- T_28956649_380000;220000;110000_Schwandorf/LConn3 -- Schwandorf___Etzenricht_CN_29084374_380000_CN_28956649_380000/RConn3
  G_129989100_Kavernenkraftwerk_Säckingen/RConn1 -- Öldruckkabel_CN_202865176_220000_CN129989100/RConn1
  G_129989100_Kavernenkraftwerk_Säckingen/RConn2 -- Öldruckkabel_CN_202865176_220000_CN129989100/RConn2
  G_129989100_Kavernenkraftwerk_Säckingen/RConn3 -- Öldruckkabel_CN_202865176_220000_CN129989100/RConn3
  T_24462228_220000;110000_Station_Ossenberg/LConn1 -- 220kV_Wesel_Ost_CN_24462426_220000_CN_24462228_220000/RConn1
  T_24462228_220000;110000_Station_Ossenberg/LConn2 -- 220kV_Wesel_Ost_CN_24462426_220000_CN_24462228_220000/RConn2
  T_24462228_220000;110000_Station_Ossenberg/LConn3 -- 220kV_Wesel_Ost_CN_24462426_220000_CN_24462228_220000/RConn3
  T_23084417_220000;110000_Station_Pfalzdorf/LConn1 -- _CN_24462426_220000_CN_23084417_220000/RConn1
  T_23084417_220000;110000_Station_Pfalzdorf/LConn2 -- _CN_24462426_220000_CN_23084417_220000/RConn2
  T_23084417_220000;110000_Station_Pfalzdorf/LConn3 -- _CN_24462426_220000_CN_23084417_220000/RConn3
  _CN_24462426_380000_CN401873466/RConn1 -- G_401873466_Kraftwerk_Voerde/RConn1 -- _CN_24479003_380000_CN401873466/LConn1 -- _CN_24479003_220000_CN401873466/LConn1 -- 380kV_Voerde_B_CN_76185022_380000_CN401873466/LConn1
  _CN_24462426_380000_CN401873466/RConn2 -- G_401873466_Kraftwerk_Voerde/RConn2 -- _CN_24479003_380000_CN401873466/LConn2 -- _CN_24479003_220000_CN401873466/LConn2 -- 380kV_Voerde_B_CN_76185022_380000_CN401873466/LConn2
  _CN_24462426_380000_CN401873466/RConn3 -- G_401873466_Kraftwerk_Voerde/RConn3 -- _CN_24479003_380000_CN401873466/LConn3 -- _CN_24479003_220000_CN401873466/LConn3 -- 380kV_Voerde_B_CN_76185022_380000_CN401873466/LConn3
  Leitung_2008_CN_33042984_220000_CN-2022229/RConn1 -- T_33042984_220000;110000_TenneT_TSO_GmbH___Betriebszentrum_Lehrte/LConn1 -- Leitung_2026_CN_33042984_220000_CN23681460/RConn1 -- _CN_33042984_220000_CN_160093341_220000/LConn1 -- _CN_33042984_220000_CN_43072656_220000/LConn1 -- _CN_33042984_220000_CN_30109913_220000/LConn1
  Leitung_2008_CN_33042984_220000_CN-2022229/RConn2 -- T_33042984_220000;110000_TenneT_TSO_GmbH___Betriebszentrum_Lehrte/LConn2 -- Leitung_2026_CN_33042984_220000_CN23681460/RConn2 -- _CN_33042984_220000_CN_160093341_220000/LConn2 -- _CN_33042984_220000_CN_43072656_220000/LConn2 -- _CN_33042984_220000_CN_30109913_220000/LConn2
  Leitung_2008_CN_33042984_220000_CN-2022229/RConn3 -- T_33042984_220000;110000_TenneT_TSO_GmbH___Betriebszentrum_Lehrte/LConn3 -- Leitung_2026_CN_33042984_220000_CN23681460/RConn3 -- _CN_33042984_220000_CN_160093341_220000/LConn3 -- _CN_33042984_220000_CN_43072656_220000/LConn3 -- _CN_33042984_220000_CN_30109913_220000/LConn3
  T_160093341_220000_Erzhausen/LConn1 -- _CN_33042984_220000_CN_160093341_220000/RConn1
  T_160093341_220000_Erzhausen/LConn2 -- _CN_33042984_220000_CN_160093341_220000/RConn2
  T_160093341_220000_Erzhausen/LConn3 -- _CN_33042984_220000_CN_160093341_220000/RConn3
  _CN_33042984_220000_CN_43072656_220000/RConn1 -- T_43072656_220000;110000_Hardegsen/LConn1 -- Leitung_2014_CN_43072656_220000_CN_29103809_220000/LConn1
  _CN_33042984_220000_CN_43072656_220000/RConn2 -- T_43072656_220000;110000_Hardegsen/LConn2 -- Leitung_2014_CN_43072656_220000_CN_29103809_220000/LConn2
  _CN_33042984_220000_CN_43072656_220000/RConn3 -- T_43072656_220000;110000_Hardegsen/LConn3 -- Leitung_2014_CN_43072656_220000_CN_29103809_220000/LConn3
  T_30109913_220000;110000_Godenau/LConn1 -- _CN_33042984_220000_CN_30109913_220000/RConn1
  T_30109913_220000;110000_Godenau/LConn2 -- _CN_33042984_220000_CN_30109913_220000/RConn2
  T_30109913_220000;110000_Godenau/LConn3 -- _CN_33042984_220000_CN_30109913_220000/RConn3
  T_202580524_380000_/LConn1 -- 380kV_Westfalen_D+E_CN_202580524_380000_CN_42488850_380000/RConn1
  T_202580524_380000_/LConn2 -- 380kV_Westfalen_D+E_CN_202580524_380000_CN_42488850_380000/RConn2
  T_202580524_380000_/LConn3 -- 380kV_Westfalen_D+E_CN_202580524_380000_CN_42488850_380000/RConn3
  T_285823537__/LConn1 -- _CN_285823537_220000_CN_22973070_220000/RConn1
  T_285823537__/LConn2 -- _CN_285823537_220000_CN_22973070_220000/RConn2
  T_285823537__/LConn3 -- _CN_285823537_220000_CN_22973070_220000/RConn3
  G_31023006_/RConn1 -- _CN_88945213_380000_CN31023006/RConn1
  G_31023006_/RConn2 -- _CN_88945213_380000_CN31023006/RConn2
  G_31023006_/RConn3 -- _CN_88945213_380000_CN31023006/RConn3
  T_31019939_380000;110000_Gundremmingen/LConn1 -- _CN_88945213_380000_CN_31019939_380000/RConn1
  T_31019939_380000;110000_Gundremmingen/LConn2 -- _CN_88945213_380000_CN_31019939_380000/RConn2
  T_31019939_380000;110000_Gundremmingen/LConn3 -- _CN_88945213_380000_CN_31019939_380000/RConn3
  T_266684854_380000_Umspannwerk_Farge/LConn1 -- _CN_266684854_380000_CN313937042/RConn1
  T_266684854_380000_Umspannwerk_Farge/LConn2 -- _CN_266684854_380000_CN313937042/RConn2
  T_266684854_380000_Umspannwerk_Farge/LConn3 -- _CN_266684854_380000_CN313937042/RConn3
  220_kV_Godorf_Ost;_Olefin_West_CN_22766160_220000_CN_32148946_220000/LConn1 -- T_22766160_380000;220000;110000_Station_Sechtem/RConn1 -- 220_kV_Troisdorf_West_CN_22766160_220000_CN_22767509_220000/RConn1 -- 220_kV_Knapsack_2b_CN_22766160_220000_CN_201153704_220000/LConn1 -- 220_kV_Godorf_Ost;_Olefin_West_CN_22766160_220000_CN_23084554_220000/LConn1
  220_kV_Godorf_Ost;_Olefin_West_CN_22766160_220000_CN_32148946_220000/LConn2 -- T_22766160_380000;220000;110000_Station_Sechtem/RConn2 -- 220_kV_Troisdorf_West_CN_22766160_220000_CN_22767509_220000/RConn2 -- 220_kV_Knapsack_2b_CN_22766160_220000_CN_201153704_220000/LConn2 -- 220_kV_Godorf_Ost;_Olefin_West_CN_22766160_220000_CN_23084554_220000/LConn2
  220_kV_Godorf_Ost;_Olefin_West_CN_22766160_220000_CN_32148946_220000/LConn3 -- T_22766160_380000;220000;110000_Station_Sechtem/RConn3 -- 220_kV_Troisdorf_West_CN_22766160_220000_CN_22767509_220000/RConn3 -- 220_kV_Knapsack_2b_CN_22766160_220000_CN_201153704_220000/LConn3 -- 220_kV_Godorf_Ost;_Olefin_West_CN_22766160_220000_CN_23084554_220000/LConn3
  T_32148946_220000;110000_Station_Bollenacker/LConn1 -- 220_kV_Godorf_Ost;_Olefin_West_CN_22766160_220000_CN_32148946_220000/RConn1
  T_32148946_220000;110000_Station_Bollenacker/LConn2 -- 220_kV_Godorf_Ost;_Olefin_West_CN_22766160_220000_CN_32148946_220000/RConn2
  T_32148946_220000;110000_Station_Bollenacker/LConn3 -- 220_kV_Godorf_Ost;_Olefin_West_CN_22766160_220000_CN_32148946_220000/RConn3
  220_kV_Godorf_Ost;_Olefin_West_CN_22766160_220000_CN_23084554_220000/RConn1 -- T_23084554_220000;110000_Station_Brauweiler/LConn1 -- 220_kV_Bocklemünd_Nord|Süd_(Brauweiler)_CN_22690852_220000_CN_23084554_220000/LConn1 -- 220_kV_Rommerskirchen_Ost_CN_24839976_220000_CN_23084554_220000/RConn1
  220_kV_Godorf_Ost;_Olefin_West_CN_22766160_220000_CN_23084554_220000/RConn2 -- T_23084554_220000;110000_Station_Brauweiler/LConn2 -- 220_kV_Bocklemünd_Nord|Süd_(Brauweiler)_CN_22690852_220000_CN_23084554_220000/LConn2 -- 220_kV_Rommerskirchen_Ost_CN_24839976_220000_CN_23084554_220000/RConn2
  220_kV_Godorf_Ost;_Olefin_West_CN_22766160_220000_CN_23084554_220000/RConn3 -- T_23084554_220000;110000_Station_Brauweiler/LConn3 -- 220_kV_Bocklemünd_Nord|Süd_(Brauweiler)_CN_22690852_220000_CN_23084554_220000/LConn3 -- 220_kV_Rommerskirchen_Ost_CN_24839976_220000_CN_23084554_220000/RConn3
  380_kV_Siegtal_Nord|Süd_CN_22766160_380000_CN_152403632_380000/RConn1 -- T_22766160_380000;220000;110000_Station_Sechtem/LConn1 -- 380_kV_Sechtem_Nord|Süd;_Walberberg_West_CN_22766160_380000_CN_26593929_380000/RConn1 -- 380_kV_Ville_Ost_CN_22766160_380000_CN_22765517_380000/LConn1 -- 380_kV_Ville_Ost_CN_22766160_380000_CN_24839976_380000/RConn1 -- 380_kV_Liessem_Ost;Mittelrhein_CN_22766160_380000_CN_395847307_380000/LConn1 -- 380_kV_Liessem_Ost;Mittelrhein_CN_22766160_380000_CN_26777313_380000/LConn1
  380_kV_Siegtal_Nord|Süd_CN_22766160_380000_CN_152403632_380000/RConn2 -- T_22766160_380000;220000;110000_Station_Sechtem/LConn2 -- 380_kV_Sechtem_Nord|Süd;_Walberberg_West_CN_22766160_380000_CN_26593929_380000/RConn2 -- 380_kV_Ville_Ost_CN_22766160_380000_CN_22765517_380000/LConn2 -- 380_kV_Ville_Ost_CN_22766160_380000_CN_24839976_380000/RConn2 -- 380_kV_Liessem_Ost;Mittelrhein_CN_22766160_380000_CN_395847307_380000/LConn2 -- 380_kV_Liessem_Ost;Mittelrhein_CN_22766160_380000_CN_26777313_380000/LConn2
  380_kV_Siegtal_Nord|Süd_CN_22766160_380000_CN_152403632_380000/RConn3 -- T_22766160_380000;220000;110000_Station_Sechtem/LConn3 -- 380_kV_Sechtem_Nord|Süd;_Walberberg_West_CN_22766160_380000_CN_26593929_380000/RConn3 -- 380_kV_Ville_Ost_CN_22766160_380000_CN_22765517_380000/LConn3 -- 380_kV_Ville_Ost_CN_22766160_380000_CN_24839976_380000/RConn3 -- 380_kV_Liessem_Ost;Mittelrhein_CN_22766160_380000_CN_395847307_380000/LConn3 -- 380_kV_Liessem_Ost;Mittelrhein_CN_22766160_380000_CN_26777313_380000/LConn3
  380_kV_Ville_Ost_CN_22766160_380000_CN_22765517_380000/RConn1 -- T_22765517_380000;110000_Station_Knapsack/LConn1 -- _CN_22765517_380000_CN239364386/LConn1 -- 380_kV_Knapsack_1a_CN_201153704_380000_CN_22765517_380000/LConn1
  380_kV_Ville_Ost_CN_22766160_380000_CN_22765517_380000/RConn2 -- T_22765517_380000;110000_Station_Knapsack/LConn2 -- _CN_22765517_380000_CN239364386/LConn2 -- 380_kV_Knapsack_1a_CN_201153704_380000_CN_22765517_380000/LConn2
  380_kV_Ville_Ost_CN_22766160_380000_CN_22765517_380000/RConn3 -- T_22765517_380000;110000_Station_Knapsack/LConn3 -- _CN_22765517_380000_CN239364386/LConn3 -- 380_kV_Knapsack_1a_CN_201153704_380000_CN_22765517_380000/LConn3
  380_kV_Liessem_Ost;Mittelrhein_CN_22766160_380000_CN_395847307_380000/RConn1 -- T_395847307_380000;220000;110000_Station_Weißenthurm/LConn1 -- _CN_160584794_380000_CN_395847307_380000/LConn1
  380_kV_Liessem_Ost;Mittelrhein_CN_22766160_380000_CN_395847307_380000/RConn2 -- T_395847307_380000;220000;110000_Station_Weißenthurm/LConn2 -- _CN_160584794_380000_CN_395847307_380000/LConn2
  380_kV_Liessem_Ost;Mittelrhein_CN_22766160_380000_CN_395847307_380000/RConn3 -- T_395847307_380000;220000;110000_Station_Weißenthurm/LConn3 -- _CN_160584794_380000_CN_395847307_380000/LConn3
  T_26777313_380000;110000_Station_Ließem/LConn1 -- 380_kV_Liessem_Ost;Mittelrhein_CN_22766160_380000_CN_26777313_380000/RConn1
  T_26777313_380000;110000_Station_Ließem/LConn2 -- 380_kV_Liessem_Ost;Mittelrhein_CN_22766160_380000_CN_26777313_380000/RConn2
  T_26777313_380000;110000_Station_Ließem/LConn3 -- 380_kV_Liessem_Ost;Mittelrhein_CN_22766160_380000_CN_26777313_380000/RConn3
  220_kV_Knapsack_2b_CN_22766160_220000_CN_201153704_220000/RConn1 -- T_201153704_380000;220000_Kraftwerkschaltanlage_Knapsack_1/RConn1 -- L_201153704/LConn1
  220_kV_Knapsack_2b_CN_22766160_220000_CN_201153704_220000/RConn2 -- T_201153704_380000;220000_Kraftwerkschaltanlage_Knapsack_1/RConn2 -- L_201153704/LConn2
  220_kV_Knapsack_2b_CN_22766160_220000_CN_201153704_220000/RConn3 -- T_201153704_380000;220000_Kraftwerkschaltanlage_Knapsack_1/RConn3 -- L_201153704/LConn3
  EDS_WDL_1x_380_kV_CN_26260052_380000_CN_26403575_380000/LConn1 -- T_26260052_380000;220000;110000_EnBW_Umspannwerk_Wendlingen/LConn1 -- EDS_WDL_1x_380_kV_CN_26260052_380000_CN_30734324_380000/LConn1 -- EDS_WDL_1x_380_kV_CN_26260052_380000_CN25973419/LConn1 -- 380_kV_CN_26260052_380000_CN_25802269_380000/LConn1 -- 380_kV_CN_26260052_380000_CN_43688805_380000/RConn1 -- 380_kV_CN_26260052_380000_CN_22960899_380000/LConn1 -- 380_kV_CN_26260052_380000_CN_41389594_380000/RConn1
  EDS_WDL_1x_380_kV_CN_26260052_380000_CN_26403575_380000/LConn2 -- T_26260052_380000;220000;110000_EnBW_Umspannwerk_Wendlingen/LConn2 -- EDS_WDL_1x_380_kV_CN_26260052_380000_CN_30734324_380000/LConn2 -- EDS_WDL_1x_380_kV_CN_26260052_380000_CN25973419/LConn2 -- 380_kV_CN_26260052_380000_CN_25802269_380000/LConn2 -- 380_kV_CN_26260052_380000_CN_43688805_380000/RConn2 -- 380_kV_CN_26260052_380000_CN_22960899_380000/LConn2 -- 380_kV_CN_26260052_380000_CN_41389594_380000/RConn2
  EDS_WDL_1x_380_kV_CN_26260052_380000_CN_26403575_380000/LConn3 -- T_26260052_380000;220000;110000_EnBW_Umspannwerk_Wendlingen/LConn3 -- EDS_WDL_1x_380_kV_CN_26260052_380000_CN_30734324_380000/LConn3 -- EDS_WDL_1x_380_kV_CN_26260052_380000_CN25973419/LConn3 -- 380_kV_CN_26260052_380000_CN_25802269_380000/LConn3 -- 380_kV_CN_26260052_380000_CN_43688805_380000/RConn3 -- 380_kV_CN_26260052_380000_CN_22960899_380000/LConn3 -- 380_kV_CN_26260052_380000_CN_41389594_380000/RConn3
  T_26403575_380000;110000_EnBW_Umspannwerk_Bünzwangen/LConn1 -- EDS_WDL_1x_380_kV_CN_26260052_380000_CN_26403575_380000/RConn1
  T_26403575_380000;110000_EnBW_Umspannwerk_Bünzwangen/LConn2 -- EDS_WDL_1x_380_kV_CN_26260052_380000_CN_26403575_380000/RConn2
  T_26403575_380000;110000_EnBW_Umspannwerk_Bünzwangen/LConn3 -- EDS_WDL_1x_380_kV_CN_26260052_380000_CN_26403575_380000/RConn3
  T_30734324_380000;220000;110000_EnBW_Umspannwerk_Metzingen/LConn1 -- EDS_WDL_1x_380_kV_CN_26260052_380000_CN_30734324_380000/RConn1
  T_30734324_380000;220000;110000_EnBW_Umspannwerk_Metzingen/LConn2 -- EDS_WDL_1x_380_kV_CN_26260052_380000_CN_30734324_380000/RConn2
  T_30734324_380000;220000;110000_EnBW_Umspannwerk_Metzingen/LConn3 -- EDS_WDL_1x_380_kV_CN_26260052_380000_CN_30734324_380000/RConn3
  EDS_WDL_1x_380_kV_CN_26260052_380000_CN25973419/RConn1 -- G_25973419_Heizkraftwerk_Altbach_Deizisau/RConn1 -- AL1_EDS_380_kV_CN_48428875_380000_CN25973419/LConn1 -- AL1_BZW_380_kV_CN_37721677_380000_CN25973419/LConn1
  EDS_WDL_1x_380_kV_CN_26260052_380000_CN25973419/RConn2 -- G_25973419_Heizkraftwerk_Altbach_Deizisau/RConn2 -- AL1_EDS_380_kV_CN_48428875_380000_CN25973419/LConn2 -- AL1_BZW_380_kV_CN_37721677_380000_CN25973419/LConn2
  EDS_WDL_1x_380_kV_CN_26260052_380000_CN25973419/RConn3 -- G_25973419_Heizkraftwerk_Altbach_Deizisau/RConn3 -- AL1_EDS_380_kV_CN_48428875_380000_CN25973419/LConn3 -- AL1_BZW_380_kV_CN_37721677_380000_CN25973419/LConn3
  380_kV_CN_26260052_380000_CN_25802269_380000/RConn1 -- T_25802269_380000;220000;110000_Umspannstation_Hoheneck_Amprion/LConn1 -- _CN_25802269_380000_CN_149987048_380000/RConn1
  380_kV_CN_26260052_380000_CN_25802269_380000/RConn2 -- T_25802269_380000;220000;110000_Umspannstation_Hoheneck_Amprion/LConn2 -- _CN_25802269_380000_CN_149987048_380000/RConn2
  380_kV_CN_26260052_380000_CN_25802269_380000/RConn3 -- T_25802269_380000;220000;110000_Umspannstation_Hoheneck_Amprion/LConn3 -- _CN_25802269_380000_CN_149987048_380000/RConn3
  T_22960899_380000;110000_Umspannwerk_Mühlhausen/LConn1 -- 380_kV_CN_26260052_380000_CN_22960899_380000/RConn1
  T_22960899_380000;110000_Umspannwerk_Mühlhausen/LConn2 -- 380_kV_CN_26260052_380000_CN_22960899_380000/RConn2
  T_22960899_380000;110000_Umspannwerk_Mühlhausen/LConn3 -- 380_kV_CN_26260052_380000_CN_22960899_380000/RConn3
  T_59026005_380000;110000_Umspannwerk_Hagenwerder/LConn1 -- _CN_59026005_380000_CN_157807291_380000/RConn1
  T_59026005_380000;110000_Umspannwerk_Hagenwerder/LConn2 -- _CN_59026005_380000_CN_157807291_380000/RConn2
  T_59026005_380000;110000_Umspannwerk_Hagenwerder/LConn3 -- _CN_59026005_380000_CN_157807291_380000/RConn3
  220kV_Siegerland_West_CN_89043564_220000_CN_132814303_220000/LConn1 -- T_89043564_220000;110000_Station_Eiserfeld/LConn1 -- 220kV_Siegerland_West_CN_89043564_220000_CN_152403632_220000/LConn1
  220kV_Siegerland_West_CN_89043564_220000_CN_132814303_220000/LConn2 -- T_89043564_220000;110000_Station_Eiserfeld/LConn2 -- 220kV_Siegerland_West_CN_89043564_220000_CN_152403632_220000/LConn2
  220kV_Siegerland_West_CN_89043564_220000_CN_132814303_220000/LConn3 -- T_89043564_220000;110000_Station_Eiserfeld/LConn3 -- 220kV_Siegerland_West_CN_89043564_220000_CN_152403632_220000/LConn3
  220kV_Siegerland_West_CN_89043564_220000_CN_132814303_220000/RConn1 -- T_132814303_220000;110000_Station_Altenkleusheim/LConn1 -- 220kV_Bixterheide_Nord+Bigge_Ost_CN_51940126_220000_CN_132814303_220000/LConn1
  220kV_Siegerland_West_CN_89043564_220000_CN_132814303_220000/RConn2 -- T_132814303_220000;110000_Station_Altenkleusheim/LConn2 -- 220kV_Bixterheide_Nord+Bigge_Ost_CN_51940126_220000_CN_132814303_220000/LConn2
  220kV_Siegerland_West_CN_89043564_220000_CN_132814303_220000/RConn3 -- T_132814303_220000;110000_Station_Altenkleusheim/LConn3 -- 220kV_Bixterheide_Nord+Bigge_Ost_CN_51940126_220000_CN_132814303_220000/LConn3
  220kV_Siegerland_West_CN_89043564_220000_CN_152403632_220000/RConn1 -- T_152403632_380000;220000;110000_Station_Dauersberg/RConn1 -- 220_kV_Leuscheid_Nord+Süd_CN_152403632_220000_CN_22767509_220000/RConn1
  220kV_Siegerland_West_CN_89043564_220000_CN_152403632_220000/RConn2 -- T_152403632_380000;220000;110000_Station_Dauersberg/RConn2 -- 220_kV_Leuscheid_Nord+Süd_CN_152403632_220000_CN_22767509_220000/RConn2
  220kV_Siegerland_West_CN_89043564_220000_CN_152403632_220000/RConn3 -- T_152403632_380000;220000;110000_Station_Dauersberg/RConn3 -- 220_kV_Leuscheid_Nord+Süd_CN_152403632_220000_CN_22767509_220000/RConn3
  PULVE_OBJTT_ENGST_380_kV;_OBJTT_ENGST_380_kV;_TRSNG_WDLNG_220_kV_CN_42736239_380000_CN_26814283_380000/RConn1 -- T_26814283_380000;110000_EnBW_Umspannwerk_Oberjettingen/LConn1 -- 2x_380_kV_CN_43688805_380000_CN_26814283_380000/RConn1
  PULVE_OBJTT_ENGST_380_kV;_OBJTT_ENGST_380_kV;_TRSNG_WDLNG_220_kV_CN_42736239_380000_CN_26814283_380000/RConn2 -- T_26814283_380000;110000_EnBW_Umspannwerk_Oberjettingen/LConn2 -- 2x_380_kV_CN_43688805_380000_CN_26814283_380000/RConn2
  PULVE_OBJTT_ENGST_380_kV;_OBJTT_ENGST_380_kV;_TRSNG_WDLNG_220_kV_CN_42736239_380000_CN_26814283_380000/RConn3 -- T_26814283_380000;110000_EnBW_Umspannwerk_Oberjettingen/LConn3 -- 2x_380_kV_CN_43688805_380000_CN_26814283_380000/RConn3
  220_kV_CN_23284340_220000_CN_31718547_220000/LConn1 -- T_23284340_380000;220000;110000_Umspannwerk_Urberach/RConn1 -- 2_x_380_kV;_3_x_220_kV_CN_23284340_220000_CN_160533153_220000/LConn1 -- 2_x_380_kV;_3_x_220_kV_CN_23284340_220000_CN_274609757_220000/LConn1
  220_kV_CN_23284340_220000_CN_31718547_220000/LConn2 -- T_23284340_380000;220000;110000_Umspannwerk_Urberach/RConn2 -- 2_x_380_kV;_3_x_220_kV_CN_23284340_220000_CN_160533153_220000/LConn2 -- 2_x_380_kV;_3_x_220_kV_CN_23284340_220000_CN_274609757_220000/LConn2
  220_kV_CN_23284340_220000_CN_31718547_220000/LConn3 -- T_23284340_380000;220000;110000_Umspannwerk_Urberach/RConn3 -- 2_x_380_kV;_3_x_220_kV_CN_23284340_220000_CN_160533153_220000/LConn3 -- 2_x_380_kV;_3_x_220_kV_CN_23284340_220000_CN_274609757_220000/LConn3
  T_31718547__/LConn1 -- 220_kV_CN_23284340_220000_CN_31718547_220000/RConn1
  T_31718547__/LConn2 -- 220_kV_CN_23284340_220000_CN_31718547_220000/RConn2
  T_31718547__/LConn3 -- 220_kV_CN_23284340_220000_CN_31718547_220000/RConn3
  T_160533153_220000;110000_Beerfelden/LConn1 -- 2_x_380_kV;_3_x_220_kV_CN_23284340_220000_CN_160533153_220000/RConn1
  T_160533153_220000;110000_Beerfelden/LConn2 -- 2_x_380_kV;_3_x_220_kV_CN_23284340_220000_CN_160533153_220000/RConn2
  T_160533153_220000;110000_Beerfelden/LConn3 -- 2_x_380_kV;_3_x_220_kV_CN_23284340_220000_CN_160533153_220000/RConn3
  2_x_380_kV;_3_x_220_kV_CN_23284340_380000_CN_24685992_380000/LConn1 -- T_23284340_380000;220000;110000_Umspannwerk_Urberach/LConn1 -- 380_kV_CN_23284340_380000_CN_42372159_380000/LConn1 -- 380_kV_CN_23284340_380000_CN_42410916_380000/LConn1 -- 2_x_380_kV;_3_x_220_kV_CN_23284340_380000_CN_55730023_380000/RConn1 -- 2_x_380_kV;_3_x_220_kV_CN_23284340_380000_CN_160584794_380000/LConn1 -- 2_x_380_kV;_3_x_220_kV_CN_23284340_380000_CN_50898216_380000/LConn1 -- 2_x_380_kV;_3_x_220_kV_CN_23284340_380000_CN_38661452_380000/LConn1 -- 2_x_380_kV;_3_x_220_kV_CN_23284340_380000_CN_149987048_380000/RConn1 -- 2_x_380_kV;_3_x_220_kV_CN_23284340_380000_CN155389593/LConn1 -- 2_x_380_kV;_3_x_220_kV_CN_23284340_380000_CN_274609757_380000/LConn1
  2_x_380_kV;_3_x_220_kV_CN_23284340_380000_CN_24685992_380000/LConn2 -- T_23284340_380000;220000;110000_Umspannwerk_Urberach/LConn2 -- 380_kV_CN_23284340_380000_CN_42372159_380000/LConn2 -- 380_kV_CN_23284340_380000_CN_42410916_380000/LConn2 -- 2_x_380_kV;_3_x_220_kV_CN_23284340_380000_CN_55730023_380000/RConn2 -- 2_x_380_kV;_3_x_220_kV_CN_23284340_380000_CN_160584794_380000/LConn2 -- 2_x_380_kV;_3_x_220_kV_CN_23284340_380000_CN_50898216_380000/LConn2 -- 2_x_380_kV;_3_x_220_kV_CN_23284340_380000_CN_38661452_380000/LConn2 -- 2_x_380_kV;_3_x_220_kV_CN_23284340_380000_CN_149987048_380000/RConn2 -- 2_x_380_kV;_3_x_220_kV_CN_23284340_380000_CN155389593/LConn2 -- 2_x_380_kV;_3_x_220_kV_CN_23284340_380000_CN_274609757_380000/LConn2
  2_x_380_kV;_3_x_220_kV_CN_23284340_380000_CN_24685992_380000/LConn3 -- T_23284340_380000;220000;110000_Umspannwerk_Urberach/LConn3 -- 380_kV_CN_23284340_380000_CN_42372159_380000/LConn3 -- 380_kV_CN_23284340_380000_CN_42410916_380000/LConn3 -- 2_x_380_kV;_3_x_220_kV_CN_23284340_380000_CN_55730023_380000/RConn3 -- 2_x_380_kV;_3_x_220_kV_CN_23284340_380000_CN_160584794_380000/LConn3 -- 2_x_380_kV;_3_x_220_kV_CN_23284340_380000_CN_50898216_380000/LConn3 -- 2_x_380_kV;_3_x_220_kV_CN_23284340_380000_CN_38661452_380000/LConn3 -- 2_x_380_kV;_3_x_220_kV_CN_23284340_380000_CN_149987048_380000/RConn3 -- 2_x_380_kV;_3_x_220_kV_CN_23284340_380000_CN155389593/LConn3 -- 2_x_380_kV;_3_x_220_kV_CN_23284340_380000_CN_274609757_380000/LConn3
  T_24685992_380000;110000_Umspannstation_Bischofsheim/LConn1 -- 2_x_380_kV;_3_x_220_kV_CN_23284340_380000_CN_24685992_380000/RConn1
  T_24685992_380000;110000_Umspannstation_Bischofsheim/LConn2 -- 2_x_380_kV;_3_x_220_kV_CN_23284340_380000_CN_24685992_380000/RConn2
  T_24685992_380000;110000_Umspannstation_Bischofsheim/LConn3 -- 2_x_380_kV;_3_x_220_kV_CN_23284340_380000_CN_24685992_380000/RConn3
  2_x_380_kV;_3_x_220_kV_CN_23284340_380000_CN_160584794_380000/RConn1 -- T_160584794_380000;110000_Station_Koblenz/LConn1 -- _CN_160584794_380000_CN_395847307_380000/RConn1 -- _CN_160584794_380000_CN_149987048_380000/RConn1
  2_x_380_kV;_3_x_220_kV_CN_23284340_380000_CN_160584794_380000/RConn2 -- T_160584794_380000;110000_Station_Koblenz/LConn2 -- _CN_160584794_380000_CN_395847307_380000/RConn2 -- _CN_160584794_380000_CN_149987048_380000/RConn2
  2_x_380_kV;_3_x_220_kV_CN_23284340_380000_CN_160584794_380000/RConn3 -- T_160584794_380000;110000_Station_Koblenz/LConn3 -- _CN_160584794_380000_CN_395847307_380000/RConn3 -- _CN_160584794_380000_CN_149987048_380000/RConn3
  2_x_380_kV;_3_x_220_kV_CN_23284340_380000_CN_50898216_380000/RConn1 -- T_50898216_380000;110000_Station_Limburg/LConn1 -- 380kV_Limburg_West_CN_50898216_380000_CN_152403632_380000/RConn1
  2_x_380_kV;_3_x_220_kV_CN_23284340_380000_CN_50898216_380000/RConn2 -- T_50898216_380000;110000_Station_Limburg/LConn2 -- 380kV_Limburg_West_CN_50898216_380000_CN_152403632_380000/RConn2
  2_x_380_kV;_3_x_220_kV_CN_23284340_380000_CN_50898216_380000/RConn3 -- T_50898216_380000;110000_Station_Limburg/LConn3 -- 380kV_Limburg_West_CN_50898216_380000_CN_152403632_380000/RConn3
  T_38661452_380000;110000_Umspannwerk_Kriftel/LConn1 -- 2_x_380_kV;_3_x_220_kV_CN_23284340_380000_CN_38661452_380000/RConn1
  T_38661452_380000;110000_Umspannwerk_Kriftel/LConn2 -- 2_x_380_kV;_3_x_220_kV_CN_23284340_380000_CN_38661452_380000/RConn2
  T_38661452_380000;110000_Umspannwerk_Kriftel/LConn3 -- 2_x_380_kV;_3_x_220_kV_CN_23284340_380000_CN_38661452_380000/RConn3
  2_x_380_kV;_3_x_220_kV_CN_23284340_220000_CN_274609757_220000/RConn1 -- T_274609757_380000;220000_Biblis_A/RConn1 -- L_274609757/LConn1
  2_x_380_kV;_3_x_220_kV_CN_23284340_220000_CN_274609757_220000/RConn2 -- T_274609757_380000;220000_Biblis_A/RConn2 -- L_274609757/LConn2
  2_x_380_kV;_3_x_220_kV_CN_23284340_220000_CN_274609757_220000/RConn3 -- T_274609757_380000;220000_Biblis_A/RConn3 -- L_274609757/LConn3
  G_155389593_Kernkraftwerk_Biblis/RConn1 -- 2_x_380_kV;_3_x_220_kV_CN_23284340_380000_CN155389593/RConn1
  G_155389593_Kernkraftwerk_Biblis/RConn2 -- 2_x_380_kV;_3_x_220_kV_CN_23284340_380000_CN155389593/RConn2
  G_155389593_Kernkraftwerk_Biblis/RConn3 -- 2_x_380_kV;_3_x_220_kV_CN_23284340_380000_CN155389593/RConn3
  T_274609757_380000;220000_Biblis_A/LConn1 -- 2_x_380_kV;_3_x_220_kV_CN_23284340_380000_CN_274609757_380000/RConn1
  T_274609757_380000;220000_Biblis_A/LConn2 -- 2_x_380_kV;_3_x_220_kV_CN_23284340_380000_CN_274609757_380000/RConn2
  T_274609757_380000;220000_Biblis_A/LConn3 -- 2_x_380_kV;_3_x_220_kV_CN_23284340_380000_CN_274609757_380000/RConn3
  T_42372159_380000;110000_Karlstein/LConn1 -- 380_kV_CN_23284340_380000_CN_42372159_380000/RConn1
  T_42372159_380000;110000_Karlstein/LConn2 -- 380_kV_CN_23284340_380000_CN_42372159_380000/RConn2
  T_42372159_380000;110000_Karlstein/LConn3 -- 380_kV_CN_23284340_380000_CN_42372159_380000/RConn3
  380_kV_CN_23284340_380000_CN_42410916_380000/RConn1 -- T_42410916_380000;220000_Umspannwerk_Großkrotzenburg/LConn1 -- AS_GKRO;GKRO_GR_I;DIP_GKB_I;_II_CN_42410916_380000_CN_55069713_380000/LConn1 -- AS_GKRO;GKRO_GR_I;DIP_GKB_I;_II_CN_42410916_380000_CN_108797675_380000/RConn1 -- AS_GKRO;GKRO_GR_I;DIP_GKB_I;_II_CN_42410916_380000_CN_148446247_380000/LConn1 -- _CN_24042358_380000_CN_42410916_380000/LConn1
  380_kV_CN_23284340_380000_CN_42410916_380000/RConn2 -- T_42410916_380000;220000_Umspannwerk_Großkrotzenburg/LConn2 -- AS_GKRO;GKRO_GR_I;DIP_GKB_I;_II_CN_42410916_380000_CN_55069713_380000/LConn2 -- AS_GKRO;GKRO_GR_I;DIP_GKB_I;_II_CN_42410916_380000_CN_108797675_380000/RConn2 -- AS_GKRO;GKRO_GR_I;DIP_GKB_I;_II_CN_42410916_380000_CN_148446247_380000/LConn2 -- _CN_24042358_380000_CN_42410916_380000/LConn2
  380_kV_CN_23284340_380000_CN_42410916_380000/RConn3 -- T_42410916_380000;220000_Umspannwerk_Großkrotzenburg/LConn3 -- AS_GKRO;GKRO_GR_I;DIP_GKB_I;_II_CN_42410916_380000_CN_55069713_380000/LConn3 -- AS_GKRO;GKRO_GR_I;DIP_GKB_I;_II_CN_42410916_380000_CN_108797675_380000/RConn3 -- AS_GKRO;GKRO_GR_I;DIP_GKB_I;_II_CN_42410916_380000_CN_148446247_380000/LConn3 -- _CN_24042358_380000_CN_42410916_380000/LConn3
  T_274621059_220000;110000_Mehrum_(220_kV)/LConn1 -- Mehrum_(220_kV)_CN_274621059_220000_CN23681460/RConn1
  T_274621059_220000;110000_Mehrum_(220_kV)/LConn2 -- Mehrum_(220_kV)_CN_274621059_220000_CN23681460/RConn2
  T_274621059_220000;110000_Mehrum_(220_kV)/LConn3 -- Mehrum_(220_kV)_CN_274621059_220000_CN23681460/RConn3
  T_46584363_380000;220000;110000_Umspannwerk_Wiesloch/LConn1 -- Elsenz_CN_143903369_380000_CN_46584363_380000/RConn1
  T_46584363_380000;220000;110000_Umspannwerk_Wiesloch/LConn2 -- Elsenz_CN_143903369_380000_CN_46584363_380000/RConn2
  T_46584363_380000;220000;110000_Umspannwerk_Wiesloch/LConn3 -- Elsenz_CN_143903369_380000_CN_46584363_380000/RConn3
  T_207248812_380000;220000_Umspannwerk_Neurott/LConn1 -- Elsenz_CN_143903369_380000_CN_207248812_380000/RConn1
  T_207248812_380000;220000_Umspannwerk_Neurott/LConn2 -- Elsenz_CN_143903369_380000_CN_207248812_380000/RConn2
  T_207248812_380000;220000_Umspannwerk_Neurott/LConn3 -- Elsenz_CN_143903369_380000_CN_207248812_380000/RConn3
  380kV_Mengede_Nord+Süd_CN_121199242_380000_CN109504648/LConn1 -- T_121199242_380000_Station_Lippe/LConn1 -- 380kV_Waltrop_Süd_CN_121199242_380000_CN4670340/LConn1 -- 380kV_Waltrop_Süd_CN_121199242_380000_CN_42507488_380000/RConn1 -- 380kV_Stummhafen_1A_CN_121199242_380000_CN109505608/LConn1 -- 380kV_Mengede_Nord+Süd_CN_121199242_380000_CN_32472806_380000/RConn1
  380kV_Mengede_Nord+Süd_CN_121199242_380000_CN109504648/LConn2 -- T_121199242_380000_Station_Lippe/LConn2 -- 380kV_Waltrop_Süd_CN_121199242_380000_CN4670340/LConn2 -- 380kV_Waltrop_Süd_CN_121199242_380000_CN_42507488_380000/RConn2 -- 380kV_Stummhafen_1A_CN_121199242_380000_CN109505608/LConn2 -- 380kV_Mengede_Nord+Süd_CN_121199242_380000_CN_32472806_380000/RConn2
  380kV_Mengede_Nord+Süd_CN_121199242_380000_CN109504648/LConn3 -- T_121199242_380000_Station_Lippe/LConn3 -- 380kV_Waltrop_Süd_CN_121199242_380000_CN4670340/LConn3 -- 380kV_Waltrop_Süd_CN_121199242_380000_CN_42507488_380000/RConn3 -- 380kV_Stummhafen_1A_CN_121199242_380000_CN109505608/LConn3 -- 380kV_Mengede_Nord+Süd_CN_121199242_380000_CN_32472806_380000/RConn3
  380kV_Mengede_Nord+Süd_CN_121199242_380000_CN109504648/RConn1 -- G_109504648_Kraftwerk_Datteln_4/RConn1 -- _CN_275138524_380000_CN109504648/LConn1
  380kV_Mengede_Nord+Süd_CN_121199242_380000_CN109504648/RConn2 -- G_109504648_Kraftwerk_Datteln_4/RConn2 -- _CN_275138524_380000_CN109504648/LConn2
  380kV_Mengede_Nord+Süd_CN_121199242_380000_CN109504648/RConn3 -- G_109504648_Kraftwerk_Datteln_4/RConn3 -- _CN_275138524_380000_CN109504648/LConn3
  G_4670340_Kraftwerk_Bergkamen/RConn1 -- 380kV_Waltrop_Süd_CN_121199242_380000_CN4670340/RConn1
  G_4670340_Kraftwerk_Bergkamen/RConn2 -- 380kV_Waltrop_Süd_CN_121199242_380000_CN4670340/RConn2
  G_4670340_Kraftwerk_Bergkamen/RConn3 -- 380kV_Waltrop_Süd_CN_121199242_380000_CN4670340/RConn3
  G_109505608_Trianel_Kraftwerk_Lünen/RConn1 -- 380kV_Stummhafen_1A_CN_121199242_380000_CN109505608/RConn1
  G_109505608_Trianel_Kraftwerk_Lünen/RConn2 -- 380kV_Stummhafen_1A_CN_121199242_380000_CN109505608/RConn2
  G_109505608_Trianel_Kraftwerk_Lünen/RConn3 -- 380kV_Stummhafen_1A_CN_121199242_380000_CN109505608/RConn3
  _CN_22973070_380000_CN_30954714_380000/RConn1 -- T_30954714_380000;110000_Umspannwerk_Friedrichshain/LConn1 -- 380_kV_Transversale_Berlin_CN_30954714_380000_CN_30303506_380000/LConn1
  _CN_22973070_380000_CN_30954714_380000/RConn2 -- T_30954714_380000;110000_Umspannwerk_Friedrichshain/LConn2 -- 380_kV_Transversale_Berlin_CN_30954714_380000_CN_30303506_380000/LConn2
  _CN_22973070_380000_CN_30954714_380000/RConn3 -- T_30954714_380000;110000_Umspannwerk_Friedrichshain/LConn3 -- 380_kV_Transversale_Berlin_CN_30954714_380000_CN_30303506_380000/LConn3
  T_26593935_380000_Station_Hambach/LConn1 -- _CN_26593935_380000_CN_26593929_380000/RConn1
  T_26593935_380000_Station_Hambach/LConn2 -- _CN_26593935_380000_CN_26593929_380000/RConn2
  T_26593935_380000_Station_Hambach/LConn3 -- _CN_26593935_380000_CN_26593929_380000/RConn3
  220kV_Neurath_1a+Osterath_West_CN_24799890_220000_CN_27919734_220000/RConn1 -- T_27919734_220000;110000_Station_Gohrpunkt/LConn1 -- 220_kV_Neurath_1a_CN_27919734_220000_CN31783693/RConn1 -- 220_kV_Neurath_1a_CN_27919734_220000_CN24267119/RConn1 -- 220_kV_Frixheim_Süd;_Zons_Nord_CN_-1897787_220000_CN_27919734_220000/RConn1 -- 220_kV_Frixheim_Nord|Süd_CN_24839976_220000_CN_27919734_220000/RConn1
  220kV_Neurath_1a+Osterath_West_CN_24799890_220000_CN_27919734_220000/RConn2 -- T_27919734_220000;110000_Station_Gohrpunkt/LConn2 -- 220_kV_Neurath_1a_CN_27919734_220000_CN31783693/RConn2 -- 220_kV_Neurath_1a_CN_27919734_220000_CN24267119/RConn2 -- 220_kV_Frixheim_Süd;_Zons_Nord_CN_-1897787_220000_CN_27919734_220000/RConn2 -- 220_kV_Frixheim_Nord|Süd_CN_24839976_220000_CN_27919734_220000/RConn2
  220kV_Neurath_1a+Osterath_West_CN_24799890_220000_CN_27919734_220000/RConn3 -- T_27919734_220000;110000_Station_Gohrpunkt/LConn3 -- 220_kV_Neurath_1a_CN_27919734_220000_CN31783693/RConn3 -- 220_kV_Neurath_1a_CN_27919734_220000_CN24267119/RConn3 -- 220_kV_Frixheim_Süd;_Zons_Nord_CN_-1897787_220000_CN_27919734_220000/RConn3 -- 220_kV_Frixheim_Nord|Süd_CN_24839976_220000_CN_27919734_220000/RConn3
  T_35818134_220000;110000_Station_Ruhrort/LConn1 -- Stockum_Ost+West_CN_35818134_220000_CN_35818137_220000/RConn1
  T_35818134_220000;110000_Station_Ruhrort/LConn2 -- Stockum_Ost+West_CN_35818134_220000_CN_35818137_220000/RConn2
  T_35818134_220000;110000_Station_Ruhrort/LConn3 -- Stockum_Ost+West_CN_35818134_220000_CN_35818137_220000/RConn3
  T_35818522_220000_/LConn1 -- _CN_35818137_220000_CN_35818522_220000/RConn1
  T_35818522_220000_/LConn2 -- _CN_35818137_220000_CN_35818522_220000/RConn2
  T_35818522_220000_/LConn3 -- _CN_35818137_220000_CN_35818522_220000/RConn3
  _CN_66038431_220000_CN_24667346_220000/LConn1 -- T_66038431_220000;110000_Station_Laer/LConn1 -- _CN_66038431_220000_CN131986820/LConn1 -- _CN_66038431_220000_CN_113546939_220000/RConn1 -- _CN_66038431_220000_CN_28452784_220000/RConn1
  _CN_66038431_220000_CN_24667346_220000/LConn2 -- T_66038431_220000;110000_Station_Laer/LConn2 -- _CN_66038431_220000_CN131986820/LConn2 -- _CN_66038431_220000_CN_113546939_220000/RConn2 -- _CN_66038431_220000_CN_28452784_220000/RConn2
  _CN_66038431_220000_CN_24667346_220000/LConn3 -- T_66038431_220000;110000_Station_Laer/LConn3 -- _CN_66038431_220000_CN131986820/LConn3 -- _CN_66038431_220000_CN_113546939_220000/RConn3 -- _CN_66038431_220000_CN_28452784_220000/RConn3
  _CN_66038431_220000_CN_24667346_220000/RConn1 -- T_24667346_220000;110000_Umspannwerk_Garenfeld/LConn1 -- 220kV_Bixterheide_Nord+Bigge_Ost_CN_51940126_220000_CN_24667346_220000/LConn1 -- 220kV_Nordleitung_CN_24667346_220000_CN_83916207_220000/LConn1
  _CN_66038431_220000_CN_24667346_220000/RConn2 -- T_24667346_220000;110000_Umspannwerk_Garenfeld/LConn2 -- 220kV_Bixterheide_Nord+Bigge_Ost_CN_51940126_220000_CN_24667346_220000/LConn2 -- 220kV_Nordleitung_CN_24667346_220000_CN_83916207_220000/LConn2
  _CN_66038431_220000_CN_24667346_220000/RConn3 -- T_24667346_220000;110000_Umspannwerk_Garenfeld/LConn3 -- 220kV_Bixterheide_Nord+Bigge_Ost_CN_51940126_220000_CN_24667346_220000/LConn3 -- 220kV_Nordleitung_CN_24667346_220000_CN_83916207_220000/LConn3
  G_131986820_Koepchenwerk/RConn1 -- _CN_66038431_220000_CN131986820/RConn1
  G_131986820_Koepchenwerk/RConn2 -- _CN_66038431_220000_CN131986820/RConn2
  G_131986820_Koepchenwerk/RConn3 -- _CN_66038431_220000_CN131986820/RConn3
  T_39688875_220000_Umspannwerk_Windpark_Iven/LConn1 -- 316_CN_39688875_220000_CN_39437430_220000/LConn1
  T_39688875_220000_Umspannwerk_Windpark_Iven/LConn2 -- 316_CN_39688875_220000_CN_39437430_220000/LConn2
  T_39688875_220000_Umspannwerk_Windpark_Iven/LConn3 -- 316_CN_39688875_220000_CN_39437430_220000/LConn3
  316_CN_39688875_220000_CN_39437430_220000/RConn1 -- T_39437430_220000;110000_Pasewalk/LConn1 -- 304_CN_39428980_220000_CN_39437430_220000/LConn1
  316_CN_39688875_220000_CN_39437430_220000/RConn2 -- T_39437430_220000;110000_Pasewalk/LConn2 -- 304_CN_39428980_220000_CN_39437430_220000/LConn2
  316_CN_39688875_220000_CN_39437430_220000/RConn3 -- T_39437430_220000;110000_Pasewalk/LConn3 -- 304_CN_39428980_220000_CN_39437430_220000/LConn3
  _CN_32318130_220000_CN_29389718_220000/LConn1 -- T_32318130_220000;110000_Bentwisch/LConn1 -- _CN_32318130_220000_CN_32062544_220000/RConn1
  _CN_32318130_220000_CN_29389718_220000/LConn2 -- T_32318130_220000;110000_Bentwisch/LConn2 -- _CN_32318130_220000_CN_32062544_220000/RConn2
  _CN_32318130_220000_CN_29389718_220000/LConn3 -- T_32318130_220000;110000_Bentwisch/LConn3 -- _CN_32318130_220000_CN_32062544_220000/RConn3
  _CN_32318130_220000_CN_29389718_220000/RConn1 -- T_29389718_220000;110000_Umspannwerk_Lüdershagen/LConn1 -- 313_CN_29389718_220000_CN_29877599_220000/LConn1
  _CN_32318130_220000_CN_29389718_220000/RConn2 -- T_29389718_220000;110000_Umspannwerk_Lüdershagen/LConn2 -- 313_CN_29389718_220000_CN_29877599_220000/LConn2
  _CN_32318130_220000_CN_29389718_220000/RConn3 -- T_29389718_220000;110000_Umspannwerk_Lüdershagen/LConn3 -- 313_CN_29389718_220000_CN_29877599_220000/LConn3
  Raitersaich___Trennfeld;Trennfeld___Aschaffenburg_CN_24765111_220000_CN_133349218_220000/LConn1 -- T_24765111_220000;110000_Umspannwerk_Trennfeld/LConn1 -- Raitersaich___Trennfeld;Trennfeld___Aschaffenburg_CN_24765111_220000_CN_55069713_220000/LConn1 -- Raitersaich___Trennfeld;Trennfeld___Aschaffenburg_CN_24765111_220000_CN_24705761_220000/RConn1
  Raitersaich___Trennfeld;Trennfeld___Aschaffenburg_CN_24765111_220000_CN_133349218_220000/LConn2 -- T_24765111_220000;110000_Umspannwerk_Trennfeld/LConn2 -- Raitersaich___Trennfeld;Trennfeld___Aschaffenburg_CN_24765111_220000_CN_55069713_220000/LConn2 -- Raitersaich___Trennfeld;Trennfeld___Aschaffenburg_CN_24765111_220000_CN_24705761_220000/RConn2
  Raitersaich___Trennfeld;Trennfeld___Aschaffenburg_CN_24765111_220000_CN_133349218_220000/LConn3 -- T_24765111_220000;110000_Umspannwerk_Trennfeld/LConn3 -- Raitersaich___Trennfeld;Trennfeld___Aschaffenburg_CN_24765111_220000_CN_55069713_220000/LConn3 -- Raitersaich___Trennfeld;Trennfeld___Aschaffenburg_CN_24765111_220000_CN_24705761_220000/RConn3
  Raitersaich___Trennfeld;Trennfeld___Aschaffenburg_CN_24765111_220000_CN_133349218_220000/RConn1 -- T_133349218_220000;110000_Umspannwerk_Ludersheim/LConn1 -- Ludersheim___Schwandorf_CN_133349218_220000_CN_28956649_220000/RConn1 -- LU_SIT_CN_24759324_220000_CN_133349218_220000/LConn1
  Raitersaich___Trennfeld;Trennfeld___Aschaffenburg_CN_24765111_220000_CN_133349218_220000/RConn2 -- T_133349218_220000;110000_Umspannwerk_Ludersheim/LConn2 -- Ludersheim___Schwandorf_CN_133349218_220000_CN_28956649_220000/RConn2 -- LU_SIT_CN_24759324_220000_CN_133349218_220000/LConn2
  Raitersaich___Trennfeld;Trennfeld___Aschaffenburg_CN_24765111_220000_CN_133349218_220000/RConn3 -- T_133349218_220000;110000_Umspannwerk_Ludersheim/LConn3 -- Ludersheim___Schwandorf_CN_133349218_220000_CN_28956649_220000/RConn3 -- LU_SIT_CN_24759324_220000_CN_133349218_220000/LConn3
  Raitersaich___Trennfeld;Trennfeld___Aschaffenburg_CN_24765111_220000_CN_55069713_220000/RConn1 -- T_55069713_380000;220000;110000_Umspannwerk_Aschaffenburg/RConn1 -- 2205;III;IIII_CN_55069713_220000_CN145861680/RConn1
  Raitersaich___Trennfeld;Trennfeld___Aschaffenburg_CN_24765111_220000_CN_55069713_220000/RConn2 -- T_55069713_380000;220000;110000_Umspannwerk_Aschaffenburg/RConn2 -- 2205;III;IIII_CN_55069713_220000_CN145861680/RConn2
  Raitersaich___Trennfeld;Trennfeld___Aschaffenburg_CN_24765111_220000_CN_55069713_220000/RConn3 -- T_55069713_380000;220000;110000_Umspannwerk_Aschaffenburg/RConn3 -- 2205;III;IIII_CN_55069713_220000_CN145861680/RConn3
  T_109917397_380000_Freiberg_Nord_(380_kV)/LConn1 -- Schmölln___Dresden_Süd___Röhrsdorf_CN_157807291_380000_CN_109917397_380000/RConn1
  T_109917397_380000_Freiberg_Nord_(380_kV)/LConn2 -- Schmölln___Dresden_Süd___Röhrsdorf_CN_157807291_380000_CN_109917397_380000/RConn2
  T_109917397_380000_Freiberg_Nord_(380_kV)/LConn3 -- Schmölln___Dresden_Süd___Röhrsdorf_CN_157807291_380000_CN_109917397_380000/RConn3
  T_23241863_380000;110000_Umspannwerk_DD_Süd/LConn1 -- Schmölln___Dresden_Süd___Röhrsdorf_CN_157807291_380000_CN_23241863_380000/RConn1
  T_23241863_380000;110000_Umspannwerk_DD_Süd/LConn2 -- Schmölln___Dresden_Süd___Röhrsdorf_CN_157807291_380000_CN_23241863_380000/RConn2
  T_23241863_380000;110000_Umspannwerk_DD_Süd/LConn3 -- Schmölln___Dresden_Süd___Röhrsdorf_CN_157807291_380000_CN_23241863_380000/RConn3
  Leitung_3018_CN_24604789_380000_CN_24230738_380000/RConn1 -- T_24230738_380000;110000_Eickum/LConn1 -- _CN_24230738_380000_CN_24264701_380000/LConn1
  Leitung_3018_CN_24604789_380000_CN_24230738_380000/RConn2 -- T_24230738_380000;110000_Eickum/LConn2 -- _CN_24230738_380000_CN_24264701_380000/LConn2
  Leitung_3018_CN_24604789_380000_CN_24230738_380000/RConn3 -- T_24230738_380000;110000_Eickum/LConn3 -- _CN_24230738_380000_CN_24264701_380000/LConn3
  _CN_26383042_380000_CN_24264701_380000/RConn1 -- T_24264701_380000;220000;110000_Umspannwerk_Bechterdissen/LConn1 -- _CN_24230738_380000_CN_24264701_380000/RConn1 -- _CN_25943440_380000_CN_24264701_380000/RConn1
  _CN_26383042_380000_CN_24264701_380000/RConn2 -- T_24264701_380000;220000;110000_Umspannwerk_Bechterdissen/LConn2 -- _CN_24230738_380000_CN_24264701_380000/RConn2 -- _CN_25943440_380000_CN_24264701_380000/RConn2
  _CN_26383042_380000_CN_24264701_380000/RConn3 -- T_24264701_380000;220000;110000_Umspannwerk_Bechterdissen/LConn3 -- _CN_24230738_380000_CN_24264701_380000/RConn3 -- _CN_25943440_380000_CN_24264701_380000/RConn3
  T_31762305_220000;110000_Station_Norf/LConn1 -- 220_kV_Frimmersdorf_5e;_Zons_Nord_CN_-1897787_220000_CN_31762305_220000/RConn1
  T_31762305_220000;110000_Station_Norf/LConn2 -- 220_kV_Frimmersdorf_5e;_Zons_Nord_CN_-1897787_220000_CN_31762305_220000/RConn2
  T_31762305_220000;110000_Station_Norf/LConn3 -- 220_kV_Frimmersdorf_5e;_Zons_Nord_CN_-1897787_220000_CN_31762305_220000/RConn3
  T_90109304_220000_UA_Dillinger_Hütte_Mitte/LConn1 -- _CN_82310607_220000_CN_90109304_220000/RConn1
  T_90109304_220000_UA_Dillinger_Hütte_Mitte/LConn2 -- _CN_82310607_220000_CN_90109304_220000/RConn2
  T_90109304_220000_UA_Dillinger_Hütte_Mitte/LConn3 -- _CN_82310607_220000_CN_90109304_220000/RConn3
  Irsching___Raitersaich_CN_24705761_380000_CN_24768051_380000/RConn1 -- T_24768051_380000;220000;110000_Ingolstadt/LConn1 -- Irsching___Raitersaich_CN_137602559_380000_CN_24768051_380000/RConn1
  Irsching___Raitersaich_CN_24705761_380000_CN_24768051_380000/RConn2 -- T_24768051_380000;220000;110000_Ingolstadt/LConn2 -- Irsching___Raitersaich_CN_137602559_380000_CN_24768051_380000/RConn2
  Irsching___Raitersaich_CN_24705761_380000_CN_24768051_380000/RConn3 -- T_24768051_380000;220000;110000_Ingolstadt/LConn3 -- Irsching___Raitersaich_CN_137602559_380000_CN_24768051_380000/RConn3
  Tiengen___Stockach_CN_31367936_220000_CN_102743264_220000/LConn1 -- T_31367936_220000;110000_Umspannwerk_Stockach/LConn1 -- Tiengen___Stockach_CN_31367936_220000_CN_31367937_220000/LConn1
  Tiengen___Stockach_CN_31367936_220000_CN_102743264_220000/LConn2 -- T_31367936_220000;110000_Umspannwerk_Stockach/LConn2 -- Tiengen___Stockach_CN_31367936_220000_CN_31367937_220000/LConn2
  Tiengen___Stockach_CN_31367936_220000_CN_102743264_220000/LConn3 -- T_31367936_220000;110000_Umspannwerk_Stockach/LConn3 -- Tiengen___Stockach_CN_31367936_220000_CN_31367937_220000/LConn3
  T_102743264_220000;110000_Beuren/LConn1 -- Tiengen___Stockach_CN_31367936_220000_CN_102743264_220000/RConn1
  T_102743264_220000;110000_Beuren/LConn2 -- Tiengen___Stockach_CN_31367936_220000_CN_102743264_220000/RConn2
  T_102743264_220000;110000_Beuren/LConn3 -- Tiengen___Stockach_CN_31367936_220000_CN_102743264_220000/RConn3
  Tiengen___Stockach_CN_31367936_220000_CN_31367937_220000/RConn1 -- T_31367937_220000;110000_Umspannwerk_Gurtweil/LConn1 -- Tiengen___Schlücht_1x_220_kV_CN_31367937_220000_CN_31367940_220000/LConn1 -- _CN_31367937_220000_CN_87653464_220000/RConn1
  Tiengen___Stockach_CN_31367936_220000_CN_31367937_220000/RConn2 -- T_31367937_220000;110000_Umspannwerk_Gurtweil/LConn2 -- Tiengen___Schlücht_1x_220_kV_CN_31367937_220000_CN_31367940_220000/LConn2 -- _CN_31367937_220000_CN_87653464_220000/RConn2
  Tiengen___Stockach_CN_31367936_220000_CN_31367937_220000/RConn3 -- T_31367937_220000;110000_Umspannwerk_Gurtweil/LConn3 -- Tiengen___Schlücht_1x_220_kV_CN_31367937_220000_CN_31367940_220000/LConn3 -- _CN_31367937_220000_CN_87653464_220000/RConn3
  T_31367940_380000;220000;110000_Tiengen/RConn1 -- Tiengen___Schlücht_1x_220_kV_CN_31367937_220000_CN_31367940_220000/RConn1
  T_31367940_380000;220000;110000_Tiengen/RConn2 -- Tiengen___Schlücht_1x_220_kV_CN_31367937_220000_CN_31367940_220000/RConn2
  T_31367940_380000;220000;110000_Tiengen/RConn3 -- Tiengen___Schlücht_1x_220_kV_CN_31367937_220000_CN_31367940_220000/RConn3
  _CN_77697810_380000_CN23802422/RConn1 -- T_77697810_380000_Isar/LConn1 -- _CN_77697810_380000_CN_24976300_380000/LConn1
  _CN_77697810_380000_CN23802422/RConn2 -- T_77697810_380000_Isar/LConn2 -- _CN_77697810_380000_CN_24976300_380000/LConn2
  _CN_77697810_380000_CN23802422/RConn3 -- T_77697810_380000_Isar/LConn3 -- _CN_77697810_380000_CN_24976300_380000/LConn3
  T_24976300_380000;220000;110000_Umspannwerk_Pleinting/LConn1 -- _CN_77697810_380000_CN_24976300_380000/RConn1
  T_24976300_380000;220000;110000_Umspannwerk_Pleinting/LConn2 -- _CN_77697810_380000_CN_24976300_380000/RConn2
  T_24976300_380000;220000;110000_Umspannwerk_Pleinting/LConn3 -- _CN_77697810_380000_CN_24976300_380000/RConn3
  220kV_Bixterheide_Nord+Bigge_Ost_CN_51940126_220000_CN_132814303_220000/RConn1 -- T_51940126_220000;110000_Umspannwerk_Bixterheide/LConn1 -- 220kV_Bixterheide_Nord+Bigge_Ost_CN_51940126_220000_CN_156398578_220000/RConn1 -- 220kV_Bixterheide_Nord+Bigge_Ost_CN_51940126_220000_CN_24667346_220000/RConn1
  220kV_Bixterheide_Nord+Bigge_Ost_CN_51940126_220000_CN_132814303_220000/RConn2 -- T_51940126_220000;110000_Umspannwerk_Bixterheide/LConn2 -- 220kV_Bixterheide_Nord+Bigge_Ost_CN_51940126_220000_CN_156398578_220000/RConn2 -- 220kV_Bixterheide_Nord+Bigge_Ost_CN_51940126_220000_CN_24667346_220000/RConn2
  220kV_Bixterheide_Nord+Bigge_Ost_CN_51940126_220000_CN_132814303_220000/RConn3 -- T_51940126_220000;110000_Umspannwerk_Bixterheide/LConn3 -- 220kV_Bixterheide_Nord+Bigge_Ost_CN_51940126_220000_CN_156398578_220000/RConn3 -- 220kV_Bixterheide_Nord+Bigge_Ost_CN_51940126_220000_CN_24667346_220000/RConn3
  T_272646943_380000_/LConn1 -- 7563_CN_272646943_380000_CN152261126/RConn1
  T_272646943_380000_/LConn2 -- 7563_CN_272646943_380000_CN152261126/RConn2
  T_272646943_380000_/LConn3 -- 7563_CN_272646943_380000_CN152261126/RConn3
  _CN_147878692_380000_CN_153328698_380000/RConn1 -- T_147878692_380000;110000_Umrichterwerk_Neckarwestheim/LConn1 -- _CN_147878692_380000_CN177942744/LConn1
  _CN_147878692_380000_CN_153328698_380000/RConn2 -- T_147878692_380000;110000_Umrichterwerk_Neckarwestheim/LConn2 -- _CN_147878692_380000_CN177942744/LConn2
  _CN_147878692_380000_CN_153328698_380000/RConn3 -- T_147878692_380000;110000_Umrichterwerk_Neckarwestheim/LConn3 -- _CN_147878692_380000_CN177942744/LConn3
  G_177942744_/RConn1 -- _CN_147878692_380000_CN177942744/RConn1
  G_177942744_/RConn2 -- _CN_147878692_380000_CN177942744/RConn2
  G_177942744_/RConn3 -- _CN_147878692_380000_CN177942744/RConn3
  T_118928165_220000_Benteler_Stahlwerk/LConn1 -- 220kV_Benteler_CN_118928165_220000_CN_61918154_220000/RConn1
  T_118928165_220000_Benteler_Stahlwerk/LConn2 -- 220kV_Benteler_CN_118928165_220000_CN_61918154_220000/RConn2
  T_118928165_220000_Benteler_Stahlwerk/LConn3 -- 220kV_Benteler_CN_118928165_220000_CN_61918154_220000/RConn3
  T_92877610__/LConn1 -- _CN_92877610_220000_CN92877616/RConn1
  T_92877610__/LConn2 -- _CN_92877610_220000_CN92877616/RConn2
  T_92877610__/LConn3 -- _CN_92877610_220000_CN92877616/RConn3
  T_90807341_220000;110000_Umspannwerk_Kempten_Au/LConn1 -- _CN_46766896_220000_CN_90807341_220000/RConn1
  T_90807341_220000;110000_Umspannwerk_Kempten_Au/LConn2 -- _CN_46766896_220000_CN_90807341_220000/RConn2
  T_90807341_220000;110000_Umspannwerk_Kempten_Au/LConn3 -- _CN_46766896_220000_CN_90807341_220000/RConn3
  T_23907283_380000;110000_Hauptumspannwerk_Menzing/LConn1 -- OBA___MZ_CN_18629425_380000_CN_23907283_380000/RConn1
  T_23907283_380000;110000_Hauptumspannwerk_Menzing/LConn2 -- OBA___MZ_CN_18629425_380000_CN_23907283_380000/RConn2
  T_23907283_380000;110000_Hauptumspannwerk_Menzing/LConn3 -- OBA___MZ_CN_18629425_380000_CN_23907283_380000/RConn3
  T_111973179_220000;110000_Station_Münster/LConn1 -- _CN_111973179_220000_CN_42861703_220000/RConn1
  T_111973179_220000;110000_Station_Münster/LConn2 -- _CN_111973179_220000_CN_42861703_220000/RConn2
  T_111973179_220000;110000_Station_Münster/LConn3 -- _CN_111973179_220000_CN_42861703_220000/RConn3
  T_92877635__/LConn1 -- _CN_92877635_220000_CN92877616/RConn1
  T_92877635__/LConn2 -- _CN_92877635_220000_CN92877616/RConn2
  T_92877635__/LConn3 -- _CN_92877635_220000_CN92877616/RConn3
  3021_UW_Lüneburg___UW_Stadorf_CN_28343121_380000_CN_28327356_380000/RConn1 -- T_28327356_380000;110000_Lüneburg/LConn1 -- _CN_23366603_380000_CN_28327356_380000/RConn1
  3021_UW_Lüneburg___UW_Stadorf_CN_28343121_380000_CN_28327356_380000/RConn2 -- T_28327356_380000;110000_Lüneburg/LConn2 -- _CN_23366603_380000_CN_28327356_380000/RConn2
  3021_UW_Lüneburg___UW_Stadorf_CN_28343121_380000_CN_28327356_380000/RConn3 -- T_28327356_380000;110000_Lüneburg/LConn3 -- _CN_23366603_380000_CN_28327356_380000/RConn3
  202A_CN_87722999_220000_CN_28008024_220000/RConn1 -- T_87722999_380000;220000_Brokdorf/RConn1 -- 202A_CN_87722999_220000_CN_60032354_220000/LConn1 -- L_87722999/LConn1
  202A_CN_87722999_220000_CN_28008024_220000/RConn2 -- T_87722999_380000;220000_Brokdorf/RConn2 -- 202A_CN_87722999_220000_CN_60032354_220000/LConn2 -- L_87722999/LConn2
  202A_CN_87722999_220000_CN_28008024_220000/RConn3 -- T_87722999_380000;220000_Brokdorf/RConn3 -- 202A_CN_87722999_220000_CN_60032354_220000/LConn3 -- L_87722999/LConn3
  202A_CN_87722999_220000_CN_60032354_220000/RConn1 -- T_60032354_220000;110000_Itzehoe_West/LConn1 -- _CN_60032354_220000_CN55015415/LConn1
  202A_CN_87722999_220000_CN_60032354_220000/RConn2 -- T_60032354_220000;110000_Itzehoe_West/LConn2 -- _CN_60032354_220000_CN55015415/LConn2
  202A_CN_87722999_220000_CN_60032354_220000/RConn3 -- T_60032354_220000;110000_Itzehoe_West/LConn3 -- _CN_60032354_220000_CN55015415/LConn3
  _CN_29309786_380000_CN_156673636_380000/RConn1 -- T_156673636_380000;110000_Umspannwerk_Borken/LConn1 -- Leitung_3212;Leitung_3213_CN_156673636_380000_CN_41072584_380000/LConn1 -- _CN_202747445_380000_CN_156673636_380000/LConn1 -- _CN_156673636_380000_CN_156960655_380000/LConn1 -- Leitung_3212;Leitung_3213_CN_156673636_380000_CN_41232144_380000/RConn1
  _CN_29309786_380000_CN_156673636_380000/RConn2 -- T_156673636_380000;110000_Umspannwerk_Borken/LConn2 -- Leitung_3212;Leitung_3213_CN_156673636_380000_CN_41072584_380000/LConn2 -- _CN_202747445_380000_CN_156673636_380000/LConn2 -- _CN_156673636_380000_CN_156960655_380000/LConn2 -- Leitung_3212;Leitung_3213_CN_156673636_380000_CN_41232144_380000/RConn2
  _CN_29309786_380000_CN_156673636_380000/RConn3 -- T_156673636_380000;110000_Umspannwerk_Borken/LConn3 -- Leitung_3212;Leitung_3213_CN_156673636_380000_CN_41072584_380000/LConn3 -- _CN_202747445_380000_CN_156673636_380000/LConn3 -- _CN_156673636_380000_CN_156960655_380000/LConn3 -- Leitung_3212;Leitung_3213_CN_156673636_380000_CN_41232144_380000/RConn3
  _CN_29309786_380000_CN_148446247_380000/RConn1 -- T_148446247_380000;110000_UW_Dipperz/LConn1 -- AS_GKRO;GKRO_GR_I;DIP_GKB_I;_II_CN_42410916_380000_CN_148446247_380000/RConn1
  _CN_29309786_380000_CN_148446247_380000/RConn2 -- T_148446247_380000;110000_UW_Dipperz/LConn2 -- AS_GKRO;GKRO_GR_I;DIP_GKB_I;_II_CN_42410916_380000_CN_148446247_380000/RConn2
  _CN_29309786_380000_CN_148446247_380000/RConn3 -- T_148446247_380000;110000_UW_Dipperz/LConn3 -- AS_GKRO;GKRO_GR_I;DIP_GKB_I;_II_CN_42410916_380000_CN_148446247_380000/RConn3
  T_232833796_220000_/LConn1 -- _CN_232833796_220000_CN_133342285_220000/RConn1
  T_232833796_220000_/LConn2 -- _CN_232833796_220000_CN_133342285_220000/RConn2
  T_232833796_220000_/LConn3 -- _CN_232833796_220000_CN_133342285_220000/RConn3
  Leitung_2014_CN_43072656_220000_CN_29103809_220000/RConn1 -- T_29103809_220000;110000_Umspannwerk_Rosdorf/LConn1 -- Leitung_2013_CN_172997498_220000_CN_29103809_220000/LConn1
  Leitung_2014_CN_43072656_220000_CN_29103809_220000/RConn2 -- T_29103809_220000;110000_Umspannwerk_Rosdorf/LConn2 -- Leitung_2013_CN_172997498_220000_CN_29103809_220000/LConn2
  Leitung_2014_CN_43072656_220000_CN_29103809_220000/RConn3 -- T_29103809_220000;110000_Umspannwerk_Rosdorf/LConn3 -- Leitung_2013_CN_172997498_220000_CN_29103809_220000/LConn3
  T_254326606_380000;110000_Umspannwerk_Bruchsal_Kändelweg/LConn1 -- Philippsburg___Pulverdingen_CN_43688805_380000_CN_254326606_380000/RConn1
  T_254326606_380000;110000_Umspannwerk_Bruchsal_Kändelweg/LConn2 -- Philippsburg___Pulverdingen_CN_43688805_380000_CN_254326606_380000/RConn2
  T_254326606_380000;110000_Umspannwerk_Bruchsal_Kändelweg/LConn3 -- Philippsburg___Pulverdingen_CN_43688805_380000_CN_254326606_380000/RConn3
  _CN_89176939_220000_CN_151967290_220000/RConn1 -- T_89176939_220000_SA_Bauler/LConn1 -- _CN_89176939_220000_CN_89176956_220000/LConn1
  _CN_89176939_220000_CN_151967290_220000/RConn2 -- T_89176939_220000_SA_Bauler/LConn2 -- _CN_89176939_220000_CN_89176956_220000/LConn2
  _CN_89176939_220000_CN_151967290_220000/RConn3 -- T_89176939_220000_SA_Bauler/LConn3 -- _CN_89176939_220000_CN_89176956_220000/LConn3
  T_89176956_220000_Vianden/LConn1 -- _CN_89176939_220000_CN_89176956_220000/RConn1
  T_89176956_220000_Vianden/LConn2 -- _CN_89176939_220000_CN_89176956_220000/RConn2
  T_89176956_220000_Vianden/LConn3 -- _CN_89176939_220000_CN_89176956_220000/RConn3
  304_CN_39428980_220000_CN215092049/RConn1 -- T_39428980_220000;110000_Vierraden/LConn1 -- 304_CN_39428980_220000_CN_30039908_220000/LConn1 -- 304_CN_39428980_220000_CN_39437430_220000/RConn1
  304_CN_39428980_220000_CN215092049/RConn2 -- T_39428980_220000;110000_Vierraden/LConn2 -- 304_CN_39428980_220000_CN_30039908_220000/LConn2 -- 304_CN_39428980_220000_CN_39437430_220000/RConn2
  304_CN_39428980_220000_CN215092049/RConn3 -- T_39428980_220000;110000_Vierraden/LConn3 -- 304_CN_39428980_220000_CN_30039908_220000/LConn3 -- 304_CN_39428980_220000_CN_39437430_220000/RConn3
  T_30039908_380000;220000_Bertikow/LConn1 -- 304_CN_39428980_220000_CN_30039908_220000/RConn1
  T_30039908_380000;220000_Bertikow/LConn2 -- 304_CN_39428980_220000_CN_30039908_220000/RConn2
  T_30039908_380000;220000_Bertikow/LConn3 -- 304_CN_39428980_220000_CN_30039908_220000/RConn3
  _CN_24042358_380000_CN_42410916_380000/RConn1 -- T_24042358_380000;110000_Umspannwerk_Karben/LConn1 -- _CN_24042358_380000_CN_202747445_380000/LConn1 -- _CN_24042358_380000_CN_62061952_380000/LConn1
  _CN_24042358_380000_CN_42410916_380000/RConn2 -- T_24042358_380000;110000_Umspannwerk_Karben/LConn2 -- _CN_24042358_380000_CN_202747445_380000/LConn2 -- _CN_24042358_380000_CN_62061952_380000/LConn2
  _CN_24042358_380000_CN_42410916_380000/RConn3 -- T_24042358_380000;110000_Umspannwerk_Karben/LConn3 -- _CN_24042358_380000_CN_202747445_380000/LConn3 -- _CN_24042358_380000_CN_62061952_380000/LConn3
  _CN_24042358_380000_CN_202747445_380000/RConn1 -- T_202747445_380000;110000_Umspannwerk_Gießen_Nord/LConn1 -- _CN_24536211_380000_CN_202747445_380000/LConn1 -- _CN_202747445_380000_CN_156673636_380000/RConn1
  _CN_24042358_380000_CN_202747445_380000/RConn2 -- T_202747445_380000;110000_Umspannwerk_Gießen_Nord/LConn2 -- _CN_24536211_380000_CN_202747445_380000/LConn2 -- _CN_202747445_380000_CN_156673636_380000/RConn2
  _CN_24042358_380000_CN_202747445_380000/RConn3 -- T_202747445_380000;110000_Umspannwerk_Gießen_Nord/LConn3 -- _CN_24536211_380000_CN_202747445_380000/LConn3 -- _CN_202747445_380000_CN_156673636_380000/RConn3
  T_62061952_380000_Umspannwerk_Frankfurt_Südwest/LConn1 -- _CN_24042358_380000_CN_62061952_380000/RConn1
  T_62061952_380000_Umspannwerk_Frankfurt_Südwest/LConn2 -- _CN_24042358_380000_CN_62061952_380000/RConn2
  T_62061952_380000_Umspannwerk_Frankfurt_Südwest/LConn3 -- _CN_24042358_380000_CN_62061952_380000/RConn3
  Leitung_2013_CN_172997498_220000_CN_29103809_220000/RConn1 -- T_172997498_220000;110000_Sandershausen/LConn1 -- _CN_172997498_220000_CN_274630377_220000/LConn1
  Leitung_2013_CN_172997498_220000_CN_29103809_220000/RConn2 -- T_172997498_220000;110000_Sandershausen/LConn2 -- _CN_172997498_220000_CN_274630377_220000/LConn2
  Leitung_2013_CN_172997498_220000_CN_29103809_220000/RConn3 -- T_172997498_220000;110000_Sandershausen/LConn3 -- _CN_172997498_220000_CN_274630377_220000/LConn3
  T_274630377_380000;220000;110000_Umspannanlage_Würgassen/RConn1 -- _CN_172997498_220000_CN_274630377_220000/RConn1
  T_274630377_380000;220000;110000_Umspannanlage_Würgassen/RConn2 -- _CN_172997498_220000_CN_274630377_220000/RConn2
  T_274630377_380000;220000;110000_Umspannanlage_Würgassen/RConn3 -- _CN_172997498_220000_CN_274630377_220000/RConn3
  207_CN_27124619_220000_CN_33148774_220000/LConn1 -- T_27124619_220000;110000_Kiel_Süd/LConn1 -- 207_CN_27124619_220000_CN_27646106_220000/LConn1 -- _CN_27124619_220000_CN149869150/LConn1
  207_CN_27124619_220000_CN_33148774_220000/LConn2 -- T_27124619_220000;110000_Kiel_Süd/LConn2 -- 207_CN_27124619_220000_CN_27646106_220000/LConn2 -- _CN_27124619_220000_CN149869150/LConn2
  207_CN_27124619_220000_CN_33148774_220000/LConn3 -- T_27124619_220000;110000_Kiel_Süd/LConn3 -- 207_CN_27124619_220000_CN_27646106_220000/LConn3 -- _CN_27124619_220000_CN149869150/LConn3
  207_CN_27124619_220000_CN_33148774_220000/RConn1 -- T_33148774_220000;110000_Audorf/LConn1 -- _CN_87952821_220000_CN_33148774_220000/LConn1 -- _CN_28008024_220000_CN_33148774_220000/RConn1
  207_CN_27124619_220000_CN_33148774_220000/RConn2 -- T_33148774_220000;110000_Audorf/LConn2 -- _CN_87952821_220000_CN_33148774_220000/LConn2 -- _CN_28008024_220000_CN_33148774_220000/RConn2
  207_CN_27124619_220000_CN_33148774_220000/RConn3 -- T_33148774_220000;110000_Audorf/LConn3 -- _CN_87952821_220000_CN_33148774_220000/LConn3 -- _CN_28008024_220000_CN_33148774_220000/RConn3
  T_27646106_220000;110000_Umspannwerk_Kiel_West/LConn1 -- 207_CN_27124619_220000_CN_27646106_220000/RConn1
  T_27646106_220000;110000_Umspannwerk_Kiel_West/LConn2 -- 207_CN_27124619_220000_CN_27646106_220000/RConn2
  T_27646106_220000;110000_Umspannwerk_Kiel_West/LConn3 -- 207_CN_27124619_220000_CN_27646106_220000/RConn3
  G_149869150_Gemeinschaftskraftwerk_Kiel/RConn1 -- _CN_27124619_220000_CN149869150/RConn1
  G_149869150_Gemeinschaftskraftwerk_Kiel/RConn2 -- _CN_27124619_220000_CN149869150/RConn2
  G_149869150_Gemeinschaftskraftwerk_Kiel/RConn3 -- _CN_27124619_220000_CN149869150/RConn3
  T_59925390_380000;110000_Station_Karnap/LConn1 -- _CN_59925390_380000_CN_113546939_380000/RConn1
  T_59925390_380000;110000_Station_Karnap/LConn2 -- _CN_59925390_380000_CN_113546939_380000/RConn2
  T_59925390_380000;110000_Station_Karnap/LConn3 -- _CN_59925390_380000_CN_113546939_380000/RConn3
  T_30622610_380000;220000;110000_Umspannwerk_Kernkraftwerk_Brunsbüttel/RConn1 -- _CN_30622610_220000_CN55015415/LConn1
  T_30622610_380000;220000;110000_Umspannwerk_Kernkraftwerk_Brunsbüttel/RConn2 -- _CN_30622610_220000_CN55015415/LConn2
  T_30622610_380000;220000;110000_Umspannwerk_Kernkraftwerk_Brunsbüttel/RConn3 -- _CN_30622610_220000_CN55015415/LConn3
  _CN_30622610_220000_CN55015415/RConn1 -- G_55015415_Gasturbinenkraftwerk_Itzehoe/RConn1 -- _CN_60032354_220000_CN55015415/RConn1
  _CN_30622610_220000_CN55015415/RConn2 -- G_55015415_Gasturbinenkraftwerk_Itzehoe/RConn2 -- _CN_60032354_220000_CN55015415/RConn2
  _CN_30622610_220000_CN55015415/RConn3 -- G_55015415_Gasturbinenkraftwerk_Itzehoe/RConn3 -- _CN_60032354_220000_CN55015415/RConn3
  313_CN_29389718_220000_CN_29877599_220000/RConn1 -- T_29877599_380000;220000_Umspannwerk_Lubmin/RConn1 -- L_29877599/LConn1
  313_CN_29389718_220000_CN_29877599_220000/RConn2 -- T_29877599_380000;220000_Umspannwerk_Lubmin/RConn2 -- L_29877599/LConn2
  313_CN_29389718_220000_CN_29877599_220000/RConn3 -- T_29877599_380000;220000_Umspannwerk_Lubmin/RConn3 -- L_29877599/LConn3
  T_31019937_380000;220000;110000_Vöhringen_LEW/LConn1 -- _CN_31019937_380000_CN_85523877_380000/RConn1
  T_31019937_380000;220000;110000_Vöhringen_LEW/LConn2 -- _CN_31019937_380000_CN_85523877_380000/RConn2
  T_31019937_380000;220000;110000_Vöhringen_LEW/LConn3 -- _CN_31019937_380000_CN_85523877_380000/RConn3
  T_41389594_380000;220000;110000_Umspannwerk_Dellmensingen/RConn1 -- Iller_Ltg__CN_31019937_220000_CN_41389594_220000/RConn1
  T_41389594_380000;220000;110000_Umspannwerk_Dellmensingen/RConn2 -- Iller_Ltg__CN_31019937_220000_CN_41389594_220000/RConn2
  T_41389594_380000;220000;110000_Umspannwerk_Dellmensingen/RConn3 -- Iller_Ltg__CN_31019937_220000_CN_41389594_220000/RConn3
  T_193674783__/LConn1 -- _CN_42410916_220000_CN_193674783_220000/RConn1
  T_193674783__/LConn2 -- _CN_42410916_220000_CN_193674783_220000/RConn2
  T_193674783__/LConn3 -- _CN_42410916_220000_CN_193674783_220000/RConn3
  T_55069713_380000;220000;110000_Umspannwerk_Aschaffenburg/LConn1 -- AS_GKRO;GKRO_GR_I;DIP_GKB_I;_II_CN_42410916_380000_CN_55069713_380000/RConn1
  T_55069713_380000;220000;110000_Umspannwerk_Aschaffenburg/LConn2 -- AS_GKRO;GKRO_GR_I;DIP_GKB_I;_II_CN_42410916_380000_CN_55069713_380000/RConn2
  T_55069713_380000;220000;110000_Umspannwerk_Aschaffenburg/LConn3 -- AS_GKRO;GKRO_GR_I;DIP_GKB_I;_II_CN_42410916_380000_CN_55069713_380000/RConn3
  T_173112252_220000;110000_Crossen/LConn1 -- 212_Röhrsdorf___Crossen_CN_173112252_220000_CN_23117075_220000/RConn1
  T_173112252_220000;110000_Crossen/LConn2 -- 212_Röhrsdorf___Crossen_CN_173112252_220000_CN_23117075_220000/RConn2
  T_173112252_220000;110000_Crossen/LConn3 -- 212_Röhrsdorf___Crossen_CN_173112252_220000_CN_23117075_220000/RConn3
  T_23837631_380000;220000;110000_Conneforde/RConn1 -- Conneforde_220_kV_CN_23837631_220000_CN_173178563_220000/RConn1
  T_23837631_380000;220000;110000_Conneforde/RConn2 -- Conneforde_220_kV_CN_23837631_220000_CN_173178563_220000/RConn2
  T_23837631_380000;220000;110000_Conneforde/RConn3 -- Conneforde_220_kV_CN_23837631_220000_CN_173178563_220000/RConn3
  302_CN_23837631_380000_CN_32076853_380000/RConn1 -- T_32076853_380000;220000;110000_Unterweser/LConn1 -- 303_CN_44717036_380000_CN_32076853_380000/LConn1 -- _CN_32076853_380000_CN_109582315_380000/LConn1
  302_CN_23837631_380000_CN_32076853_380000/RConn2 -- T_32076853_380000;220000;110000_Unterweser/LConn2 -- 303_CN_44717036_380000_CN_32076853_380000/LConn2 -- _CN_32076853_380000_CN_109582315_380000/LConn2
  302_CN_23837631_380000_CN_32076853_380000/RConn3 -- T_32076853_380000;220000;110000_Unterweser/LConn3 -- 303_CN_44717036_380000_CN_32076853_380000/LConn3 -- _CN_32076853_380000_CN_109582315_380000/LConn3
  T_32725958_220000;110000_Karlsruhe_Rintheim/LConn1 -- _CN_32725957_220000_CN_32725958_220000/RConn1
  T_32725958_220000;110000_Karlsruhe_Rintheim/LConn2 -- _CN_32725957_220000_CN_32725958_220000/RConn2
  T_32725958_220000;110000_Karlsruhe_Rintheim/LConn3 -- _CN_32725957_220000_CN_32725958_220000/RConn3
  G_43912398_Kernkraftwerk_Emsland/RConn1 -- 380_kV_Kernkraftwerk_Emsland_CN_61918154_380000_CN43912398/RConn1
  G_43912398_Kernkraftwerk_Emsland/RConn2 -- 380_kV_Kernkraftwerk_Emsland_CN_61918154_380000_CN43912398/RConn2
  G_43912398_Kernkraftwerk_Emsland/RConn3 -- 380_kV_Kernkraftwerk_Emsland_CN_61918154_380000_CN43912398/RConn3
  _CN_61918154_380000_CN49339874/RConn1 -- G_49339874_Erdgaskraftwerk_Emsland/RConn1 -- Emsland_D1|D2|D0_CN_157449983_380000_CN49339874/LConn1
  _CN_61918154_380000_CN49339874/RConn2 -- G_49339874_Erdgaskraftwerk_Emsland/RConn2 -- Emsland_D1|D2|D0_CN_157449983_380000_CN49339874/LConn2
  _CN_61918154_380000_CN49339874/RConn3 -- G_49339874_Erdgaskraftwerk_Emsland/RConn3 -- Emsland_D1|D2|D0_CN_157449983_380000_CN49339874/LConn3
  T_23682013_220000;110000_Hannover_West/LConn1 -- 2016_CN_23682013_220000_CN-2022229/RConn1
  T_23682013_220000;110000_Hannover_West/LConn2 -- 2016_CN_23682013_220000_CN-2022229/RConn2
  T_23682013_220000;110000_Hannover_West/LConn3 -- 2016_CN_23682013_220000_CN-2022229/RConn3
  303_CN_44717036_380000_CN_24493551_380000/LConn1 -- T_44717036_380000;110000_Niedervieland/LConn1 -- 303_CN_44717036_380000_CN_32076853_380000/RConn1 -- 303_CN_44717036_380000_CN313937042/RConn1
  303_CN_44717036_380000_CN_24493551_380000/LConn2 -- T_44717036_380000;110000_Niedervieland/LConn2 -- 303_CN_44717036_380000_CN_32076853_380000/RConn2 -- 303_CN_44717036_380000_CN313937042/RConn2
  303_CN_44717036_380000_CN_24493551_380000/LConn3 -- T_44717036_380000;110000_Niedervieland/LConn3 -- 303_CN_44717036_380000_CN_32076853_380000/RConn3 -- 303_CN_44717036_380000_CN313937042/RConn3
  T_24493551_380000;110000_Ganderkesee/LConn1 -- 303_CN_44717036_380000_CN_24493551_380000/RConn1
  T_24493551_380000;110000_Ganderkesee/LConn2 -- 303_CN_44717036_380000_CN_24493551_380000/RConn2
  T_24493551_380000;110000_Ganderkesee/LConn3 -- 303_CN_44717036_380000_CN_24493551_380000/RConn3
  G_29122363_Kraftwerk_Irsching/RConn1 -- _CN_137602559_220000_CN29122363/RConn1
  G_29122363_Kraftwerk_Irsching/RConn2 -- _CN_137602559_220000_CN29122363/RConn2
  G_29122363_Kraftwerk_Irsching/RConn3 -- _CN_137602559_220000_CN29122363/RConn3
  T_40621568_220000;110000_Brandenburg_West/LConn1 -- 324_CN_40621568_220000_CN_27149550_220000/RConn1
  T_40621568_220000;110000_Brandenburg_West/LConn2 -- 324_CN_40621568_220000_CN_27149550_220000/RConn2
  T_40621568_220000;110000_Brandenburg_West/LConn3 -- 324_CN_40621568_220000_CN_27149550_220000/RConn3
  T_194446360_380000_/LConn1 -- 7564_CN_194446360_380000_CN152261126/RConn1
  T_194446360_380000_/LConn2 -- 7564_CN_194446360_380000_CN152261126/RConn2
  T_194446360_380000_/LConn3 -- 7564_CN_194446360_380000_CN152261126/RConn3
  LU_SIT_CN_24759324_220000_CN_133349218_220000/RConn1 -- T_24759324_220000;110000_Umspannwerk_Sittling/LConn1 -- Altheim___Sittling_CN_24759324_220000_CN_77694901_220000/RConn1 -- IN_SIT_CN_24759324_220000_CN_24768051_220000/LConn1
  LU_SIT_CN_24759324_220000_CN_133349218_220000/RConn2 -- T_24759324_220000;110000_Umspannwerk_Sittling/LConn2 -- Altheim___Sittling_CN_24759324_220000_CN_77694901_220000/RConn2 -- IN_SIT_CN_24759324_220000_CN_24768051_220000/LConn2
  LU_SIT_CN_24759324_220000_CN_133349218_220000/RConn3 -- T_24759324_220000;110000_Umspannwerk_Sittling/LConn3 -- Altheim___Sittling_CN_24759324_220000_CN_77694901_220000/RConn3 -- IN_SIT_CN_24759324_220000_CN_24768051_220000/LConn3
  T_24768051_380000;220000;110000_Ingolstadt/RConn1 -- IN_SIT_CN_24759324_220000_CN_24768051_220000/RConn1
  T_24768051_380000;220000;110000_Ingolstadt/RConn2 -- IN_SIT_CN_24759324_220000_CN_24768051_220000/RConn2
  T_24768051_380000;220000;110000_Ingolstadt/RConn3 -- IN_SIT_CN_24759324_220000_CN_24768051_220000/RConn3
  T_22690852_220000;110000_Bocklemünd/LConn1 -- 220_kV_Bocklemünd_Nord|Süd_(Brauweiler)_CN_22690852_220000_CN_23084554_220000/RConn1
  T_22690852_220000;110000_Bocklemünd/LConn2 -- 220_kV_Bocklemünd_Nord|Süd_(Brauweiler)_CN_22690852_220000_CN_23084554_220000/RConn2
  T_22690852_220000;110000_Bocklemünd/LConn3 -- 220_kV_Bocklemünd_Nord|Süd_(Brauweiler)_CN_22690852_220000_CN_23084554_220000/RConn3
  T_109582315_380000;220000_Kernkraftwerk_Unterweser/LConn1 -- _CN_32076853_380000_CN_109582315_380000/RConn1
  T_109582315_380000;220000_Kernkraftwerk_Unterweser/LConn2 -- _CN_32076853_380000_CN_109582315_380000/RConn2
  T_109582315_380000;220000_Kernkraftwerk_Unterweser/LConn3 -- _CN_32076853_380000_CN_109582315_380000/RConn3
  T_32076853_380000;220000;110000_Unterweser/RConn1 -- 302_CN_32076853_220000_CN_173178563_220000/RConn1
  T_32076853_380000;220000;110000_Unterweser/RConn2 -- 302_CN_32076853_220000_CN_173178563_220000/RConn2
  T_32076853_380000;220000;110000_Unterweser/RConn3 -- 302_CN_32076853_220000_CN_173178563_220000/RConn3
  G_161909939_Kernkraftwerk_Philippsburg/RConn1 -- _CN_154110135_380000_CN161909939/RConn1
  G_161909939_Kernkraftwerk_Philippsburg/RConn2 -- _CN_154110135_380000_CN161909939/RConn2
  G_161909939_Kernkraftwerk_Philippsburg/RConn3 -- _CN_154110135_380000_CN161909939/RConn3
  903;_904_CN_11500045_380000_CN_46615737_380000/LConn1 -- T_11500045_380000_380_kV_Kabel_Terminal_Berlin/LConn1 -- 903;_904_CN_11500045_380000_CN185569568/RConn1
  903;_904_CN_11500045_380000_CN_46615737_380000/LConn2 -- T_11500045_380000_380_kV_Kabel_Terminal_Berlin/LConn2 -- 903;_904_CN_11500045_380000_CN185569568/RConn2
  903;_904_CN_11500045_380000_CN_46615737_380000/LConn3 -- T_11500045_380000_380_kV_Kabel_Terminal_Berlin/LConn3 -- 903;_904_CN_11500045_380000_CN185569568/RConn3
  903;_904_CN_11500045_380000_CN_46615737_380000/RConn1 -- T_46615737_380000;110000_Umspannwerk_Charlottenburg/LConn1 -- 380_kV_Transversale_Berlin_CN_46615737_380000_CN_30303506_380000/LConn1
  903;_904_CN_11500045_380000_CN_46615737_380000/RConn2 -- T_46615737_380000;110000_Umspannwerk_Charlottenburg/LConn2 -- 380_kV_Transversale_Berlin_CN_46615737_380000_CN_30303506_380000/LConn2
  903;_904_CN_11500045_380000_CN_46615737_380000/RConn3 -- T_46615737_380000;110000_Umspannwerk_Charlottenburg/LConn3 -- 380_kV_Transversale_Berlin_CN_46615737_380000_CN_30303506_380000/LConn3
  T_176704629__/LConn1 -- _CN_176704629_220000_CN30425117/LConn1
  T_176704629__/LConn2 -- _CN_176704629_220000_CN30425117/LConn2
  T_176704629__/LConn3 -- _CN_176704629_220000_CN30425117/LConn3
  _CN_176704629_220000_CN30425117/RConn1 -- G_30425117_Kraftwerk_Weiher/RConn1 -- _CN_54359256_220000_CN30425117/RConn1 -- _CN_100812630_220000_CN30425117/LConn1
  _CN_176704629_220000_CN30425117/RConn2 -- G_30425117_Kraftwerk_Weiher/RConn2 -- _CN_54359256_220000_CN30425117/RConn2 -- _CN_100812630_220000_CN30425117/LConn2
